simulink model "RBDmodel"  (R2023a)
settings: Solver=ode15s  StartTime=0.0  StopTime=4  FixedStep=0.0001  RelTol=1e-3  AbsTol=1e-3  EnableMultiTasking=on
model workspace (MAT data in the model file):
  C_Gimbal = 0.5
  C_IAP = 0.01
  IAP_Pa = 0
  K_Gimbal = 0
  K_IAP = 200
  LeftAbdominalMuscleForce = 0
  LeftBackMuscleForce = 0
  LeftTransverse1MuscleForce = 0
  LeftTransverse2MuscleForce = 0
  Moment_AR = 0
  Moment_FE = 7.5
  Moment_LB = 0
  RightAbdominalMuscleForce = 0
  RightBackMuscleForce = 0
  RightTransverse1MuscleForce = 0
  RightTransverse2MuscleForce = 0
  a = 1
  b = 1
  muscle_color = [0 0 1]
  muscle_radius = 1
undefined symbols (not defined in the file): X, Y, Z
libraries: nesl_utility x346, sm_lib x329, simulink_extras x33, checkpacklib x3, simulink x1
(part 5 of 12)

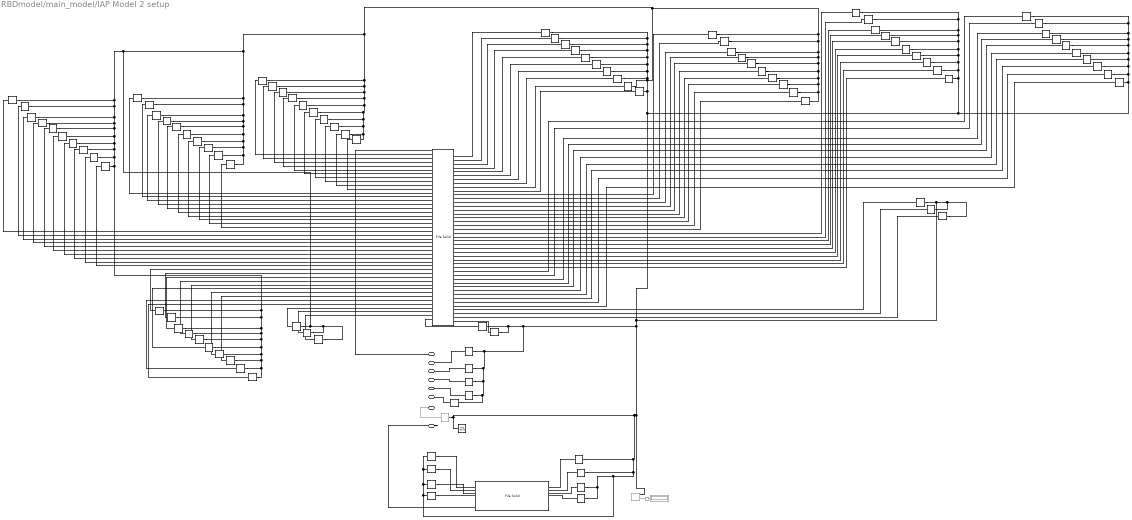
== system RBDmodel/main_model/IAP Model 2 setup ==
  Display : Display  Commented=on
  File Solid : sm_lib/Body Elements/File Solid  ExtGeomFileName=C:\Users\siril\OneDrive\Desktop\TIM-Control\Matlab\Simscape models\CAD - with COM\SymmetricModel\Abdominal COM Cone.step  UnitType=FromFile  ExtGeomFileUnits=m  StepReaderType=HEX  ExportConvexHullGeometry=off  InertiaType=CalculateFromGeometry  Mass=1  MassUnits=g  CenterOfMass=[0 0 0]  CenterOfMassUnits=m  MomentsOfInertia=[1 1 1]  MomentsOfInertiaUnits=kg*m^2  ProductsOfInertia=[0 0 0]  ProductsOfInertiaUnits=kg*m^2  BasedOnType=Density  Density=1000  DensityUnits=kg/m^3  DoExposeReferenceFrame=off  SerializedFrames=<Frames><Frame><Id>Frame1</Id><Value><Name>Abdominal COM</Name><Origin><Source>GeometricFeature</Source><FeatureName>point 8</FeatureName></Origin><PrimaryAxis><DefinedDirection>+Z</DefinedDirection><Source>ReferenceFrame</Source><SourceDirection>+Z</SourceDirection><FeatureName></FeatureName></PrimaryAxis><SecondaryAxis><DefinedDirection>+X</DefinedDirection><Source>ReferenceFrame</Source><SourceDirection>+X</SourceDirection><FeatureName></FeatureName></SecondaryAxis></Value></Frame></Frames>  GraphicType=FromGeometry  MarkerShape=Sphere  MarkerSize=10  GraphicVisPropType=SimpleVisualProperties  GraphicDiffuseColor=[1.0 0.2 0.2]  GraphicSpecularColor=[0.5 0.5 0.5 1.0]  GraphicAmbientColor=[0.15 0.15 0.15 1.0]  GraphicEmissiveColor=[0.0 0.0 0.0 1.0]  GraphicShininess=75  GraphicOpacity=1.0
  File Solid2 : sm_lib/Body Elements/File Solid  ExtGeomFileName=C:\Users\siril\OneDrive\Desktop\TIM-Control\Matlab\Simscape models\CAD - with COM\SymmetricModel\draft7\Abd-diamond-flat-solid.step  UnitType=FromFile  ExtGeomFileUnits=m  StepReaderType=HEX  ExportConvexHullGeometry=off  InertiaType=CalculateFromGeometry  Mass=1  MassUnits=kg  CenterOfMass=[0 0 0]  CenterOfMassUnits=m  MomentsOfInertia=[1 1 1]  MomentsOfInertiaUnits=kg*m^2  ProductsOfInertia=[0 0 0]  ProductsOfInertiaUnits=kg*m^2  BasedOnType=Density  Density=0.182  DensityUnits=g/cm^3  DoExposeReferenceFrame=on  SerializedFrames=<Frames><Frame><Id>Frame1</Id><Value><Name>To L1</Name><Origin><Source>GeometricFeature</Source><FeatureName>planar surface 723</FeatureName></Origin><PrimaryAxis><DefinedDirection>-Z</DefinedDirection><Source>GeometricFeature</Source><SourceDirection>+Z</SourceDirection><FeatureName>planar surface 723</FeatureName></PrimaryAxis><SecondaryAxis><DefinedDirection>+X</DefinedDirection><Source>ReferenceFrame</Source><SourceDirection>+X</SourceDirection><FeatureName></FeatureName></SecondaryAxis></Value></Frame><Frame><Id>Frame2</Id><Value><Name>L1</Name><Origin><Source>GeometricFeature</Source><FeatureName>planar surface 1442</FeatureName></Origin><PrimaryAxis><DefinedDirection>+Z</DefinedDirection><Source>GeometricFeature</Source><SourceDirection>+Z</SourceDirection><FeatureName>planar surface 1442</FeatureName></PrimaryAxis><SecondaryAxis><DefinedDirection>+X</DefinedDirection><Source>ReferenceFrame</Source><SourceDirection>+X</SourceDirection><FeatureName></FeatureName></SecondaryAxis></Value></Frame><Frame><Id>Frame3</Id><Value><Name>R1</Name><Origin><Source>GeometricFeature</Source><FeatureName>planar surface 707</FeatureName></Origin><PrimaryAxis><DefinedDirection>-Z</DefinedDirection><Source>GeometricFeature</Source><SourceDirection>+Z</SourceDirection><FeatureName>planar surface 707</FeatureName></PrimaryAxis><SecondaryAxis><DefinedDirection>+X</DefinedDirection><Source>ReferenceFrame</Source><SourceDirection>+X</SourceDirection><FeatureName></FeatureName></SecondaryAxis></Value></Frame><Frame><Id>Frame4</Id><Value><Name>L2</Name><Origin><Source>GeometricFeature</Source><FeatureName>planar surface 1450</FeatureName></Origin><PrimaryAxis><DefinedDirection>+Z</DefinedDirection><Source>GeometricFeature</Source><SourceDirection>+Z</SourceDirection><FeatureName>planar surface 1450</FeatureName></PrimaryAxis><SecondaryAxis><DefinedDirection>+X</DefinedDirection><Source>ReferenceFrame</Source><SourceDirection>+X</SourceDirection><FeatureName></FeatureName></SecondaryAxis></Value></Frame><Frame><Id>Frame5</Id><Value><Name>R2</Name><Origin><Source>GeometricFeature</Source><FeatureName>planar surface 715</FeatureName></Origin><PrimaryAxis><DefinedDirection>-Z</DefinedDirection><Source>GeometricFeature</Source><SourceDirection>+Z</SourceDirection><FeatureName>planar surface 715</FeatureName></PrimaryAxis><SecondaryAxis><DefinedDirection>+X</DefinedDirection><Source>ReferenceFrame</Source><SourceDirection>+X</SourceDirection><FeatureName></FeatureName></SecondaryAxis></Value></Frame><Frame><Id>Frame6</Id><Value><Name>L3</Name><Origin><Source>GeometricFeature</Source><FeatureName>planar surface 1412</FeatureName></Origin><PrimaryAxis><DefinedDirection>+Z</DefinedDirection><Source>GeometricFeature</Source><SourceDirection>+Z</SourceDirection><FeatureName>planar surface 1412</FeatureName></PrimaryAxis><SecondaryAxis><DefinedDirection>+X</DefinedDirection><Source>ReferenceFrame</Source><SourceDirection>+X</SourceDirection><FeatureName></FeatureName></SecondaryAxis></Value></Frame><Frame><Id>Frame7</Id><Value><Name>R3</Name><Origin><Source>GeometricFeature</Source><FeatureName>planar surface 677</FeatureName></Origin><PrimaryAxis><DefinedDirection>-Z</DefinedDirection><Source>GeometricFeature</Source><SourceDirection>+Z</SourceDirection><FeatureName>planar surface 677</FeatureName></PrimaryAxis><SecondaryAxis><DefinedDirection>+X</DefinedDirection><Source>ReferenceFrame</Source><SourceDirection>+X</SourceDirection><FeatureName></FeatureName></SecondaryAxis></Value></Frame><Frame><Id>Frame8</Id><Value><Name>L4</Name><Origin><Source>GeometricFeature</Source><FeatureName>planar surface 1159</FeatureName></Origin><PrimaryAxis><DefinedDirection>+Z</DefinedDirection><Source>GeometricFeature</Source><SourceDirection>+Z</SourceDirection><FeatureName>planar surface 1159</FeatureName></PrimaryAxis><SecondaryAxis><DefinedDirection>+X</DefinedDirection><Source>ReferenceFrame</Source><SourceDirection>+X</SourceDirection><FeatureName></FeatureName></SecondaryAxis></Value></Frame><Frame><Id>Frame9</Id><Value><Name>R4</Name><Origin><Source>GeometricFeature</Source><FeatureName>planar surface 431</FeatureName></Origin><PrimaryAxis><DefinedDirection>-Z</DefinedDirection><Source>GeometricFeature</Source><SourceDirection>+Z</SourceDirection><FeatureName>planar surface 431</FeatureName></PrimaryAxis><SecondaryAxis><DefinedDirection>+X</DefinedDirection><Source>ReferenceFrame</Source><SourceDirection>+X</SourceDirection><FeatureName></FeatureName></SecondaryAxis></Value></Frame><Frame><Id>Frame10</Id><Value><Name>L5</Name><Origin><Source>GeometricFeature</Source><FeatureName>planar surface 1433</FeatureName></Origin><PrimaryAxis><DefinedDirection>+Z</DefinedDirection><Source>GeometricFeature</Source><SourceDirection>+Z</SourceDirection><FeatureName>planar surface 1433</FeatureName></PrimaryAxis><SecondaryAxis><DefinedDirection>+X</DefinedDirection><Source>ReferenceFrame</Source><SourceDirection>+X</SourceDirection><FeatureName></FeatureName></SecondaryAxis></Value></Frame><Frame><Id>Frame11</Id><Value><Name>R5</Name><Origin><Source>GeometricFeature</Source><FeatureName>planar surface 698</FeatureName></Origin><PrimaryAxis><DefinedDirection>-Z</DefinedDirection><Source>GeometricFeature</Source><SourceDirection>+Z</SourceDirection><FeatureName>planar surface 698</FeatureName></PrimaryAxis><SecondaryAxis><DefinedDirection>+X</DefinedDirection><Source>ReferenceFrame</Source><SourceDirection>+X</SourceDirection><FeatureName></FeatureName></SecondaryAxis></Value></Frame><Frame><Id>Frame12</Id><Value><Name>L6</Name><Origin><Source>GeometricFeature</Source><FeatureName>planar surface 1135</FeatureName></Origin><PrimaryAxis><DefinedDirection>+Z</DefinedDirection><Source>GeometricFeature</Source><SourceDirection>+Z</SourceDirection><FeatureName>planar surface 1135</FeatureName></PrimaryAxis><SecondaryAxis><DefinedDirection>+X</DefinedDirection><Source>ReferenceFrame</Source><SourceDirection>+X</SourceDirection><FeatureName></FeatureName></SecondaryAxis></Value></Frame><Frame><Id>Frame13</Id><Value><Name>R6</Name><Origin><Source>GeometricFeature</Source><FeatureName>planar surface 407</FeatureName></Origin><PrimaryAxis><DefinedDirection>-Z</DefinedDirection><Source>GeometricFeature</Source><SourceDirection>+Z</SourceDirection><FeatureName>planar surface 407</FeatureName></PrimaryAxis><SecondaryAxis><DefinedDirection>+X</DefinedDirection><Source>ReferenceFrame</Source><SourceDirection>+X</SourceDirection><FeatureName></FeatureName></SecondaryAxis></Value></Frame><Frame><Id>Frame14</Id><Value><Name>L7</Name><Origin><Source>GeometricFeature</Source><FeatureName>planar surface 1217</FeatureName></Origin><PrimaryAxis><DefinedDirection>+Z</DefinedDirection><Source>GeometricFeature</Source><SourceDirection>+Z</SourceDirection><FeatureName>planar surface 1217</FeatureName></PrimaryAxis><SecondaryAxis><DefinedDirection>+X</DefinedDirection><Source>ReferenceFrame</Source><SourceDirection>+X</SourceDirection><FeatureName></FeatureName></SecondaryAxis></Value></Frame><Frame><Id>Frame15</Id><Value><Name>R7</Name><Origin><Source>GeometricFeature</Source><FeatureName>planar surface 482</FeatureName></Origin><PrimaryAxis><DefinedDirection>-Z</DefinedDirection><Source>GeometricFeature</Source><SourceDirection>+Z</SourceDirection><FeatureName>planar surface 482</FeatureName></PrimaryAxis><SecondaryAxis><DefinedDirection>+X</DefinedDirection><Source>ReferenceFrame</Source><SourceDirection>+X</SourceDirection><FeatureName></FeatureName></SecondaryAxis></Value></Frame><Frame><Id>Frame16</Id><Value><Name>L8</Name><Origin><Source>GeometricFeature</Source><FeatureName>planar surface 1125</FeatureName></Origin><PrimaryAxis><DefinedDirection>+Z</DefinedDirection><Source>GeometricFeature</Source><SourceDirection>+Z</SourceDirection><FeatureName>planar surface 1125</FeatureName></PrimaryAxis><SecondaryAxis><DefinedDirection>+X</DefinedDirection><Source>ReferenceFrame</Source><SourceDirection>+X</SourceDirection><FeatureName></FeatureName></SecondaryAxis></Value></Frame><Frame><Id>Frame17</Id><Value><Name>R8</Name><Origin><Source>GeometricFeature</Source><FeatureName>planar surface 397</FeatureName></Origin><PrimaryAxis><DefinedDirection>-Z</DefinedDirection><Source>GeometricFeature</Source><SourceDirection>+Z</SourceDirection><FeatureName>planar surface 397</FeatureName></PrimaryAxis><SecondaryAxis><DefinedDirection>+X</DefinedDirection><Source>ReferenceFrame</Source><SourceDirection>+X</SourceDirection><FeatureName></FeatureName></SecondaryAxis></Value></Frame><Frame><Id>Frame18</Id><Value><Name>L9</Name><Origin><Source>GeometricFeature</Source><FeatureName>planar surface 1123</FeatureName></Origin><PrimaryAxis><DefinedDirection>+Z</DefinedDirection><Source>GeometricFeature</Source><SourceDirection>+Z</SourceDirection><FeatureName>planar surface 1123</FeatureName></PrimaryAxis><SecondaryAxis><DefinedDirection>+X</DefinedDirection><Source>ReferenceFrame</Source><SourceDirection>+X</SourceDirection><FeatureName></FeatureName></SecondaryAxis></Value></Frame><Frame><Id>Frame19</Id><Value><Name>R9</Name><Origin><Source>GeometricFeature</Source><FeatureName>planar surface 395</FeatureName></Origin><PrimaryAxis><DefinedDirection>-Z</DefinedDirection><Source>GeometricFeature</Source><SourceDirection>+Z</SourceDirection><FeatureName>planar surface 395</FeatureName></PrimaryAxis><SecondaryAxis><DefinedDirection>+X</DefinedDirection><Source>ReferenceFrame</Source><SourceDirection>+X</SourceDirection><FeatureName></FeatureName></SecondaryAxis></Value></Frame><Frame><Id>Frame20</Id><Value><Name>L10</Name><Origin><Source>GeometricFeature</Source><FeatureName>planar surface 1120</FeatureName></Origin><PrimaryAxis><DefinedDirection>+Z</DefinedDirection><Source>GeometricFeature</Source><SourceDirection>+Z</SourceDirection><FeatureName>planar surface 1120</FeatureName></PrimaryAxis><SecondaryAxis><DefinedDirection>+X</DefinedDirection><Source>ReferenceFrame</Source><SourceDirection>+X</SourceDirection><FeatureName></FeatureName></SecondaryAxis></Value></Frame><Frame><Id>Frame21</Id><Value><Name>R10</Name><Origin><Source>GeometricFeature</Source><FeatureName>planar surface 392</FeatureName></Origin><PrimaryAxis><DefinedDirection>-Z</DefinedDirection><Source>GeometricFeature</Source><SourceDirection>+Z</SourceDirection><FeatureName>planar surface 392</FeatureName></PrimaryAxis><SecondaryAxis><DefinedDirection>+X</DefinedDirection><Source>ReferenceFrame</Source><SourceDirection>+X</SourceDirection><FeatureName></FeatureName></SecondaryAxis></Value></Frame><Frame><Id>Frame22</Id><Value><Name>L11</Name><Origin><Source>GeometricFeature</Source><FeatureName>planar surface 1182</FeatureName></Origin><PrimaryAxis><DefinedDirection>+Z</DefinedDirection><Source>GeometricFeature</Source><SourceDirection>+Z</SourceDirection><FeatureName>planar surface 1182</FeatureName></PrimaryAxis><SecondaryAxis><DefinedDirection>+X</DefinedDirection><Source>ReferenceFrame</Source><SourceDirection>+X</SourceDirection><FeatureName></FeatureName></SecondaryAxis></Value></Frame><Frame><Id>Frame23</Id><Value><Name>R11</Name><Origin><Source>GeometricFeature</Source><FeatureName>planar surface 452</FeatureName></Origin><PrimaryAxis><DefinedDirection>-Z</DefinedDirection><Source>GeometricFeature</Source><SourceDirection>+Z</SourceDirection><FeatureName>planar surface 452</FeatureName></PrimaryAxis><SecondaryAxis><DefinedDirection>+X</DefinedDirection><Source>ReferenceFrame</Source><SourceDirection>+X</SourceDirection><FeatureName></FeatureName></SecondaryAxis></Value></Frame><Frame><Id>Frame24</Id><Value><Name>L12</Name><Origin><Source>GeometricFeature</Source><FeatureName>planar surface 1305</FeatureName></Origin><PrimaryAxis><DefinedDirection>+Z</DefinedDirection><Source>GeometricFeature</Source><SourceDirection>+Z</SourceDirection><FeatureName>planar surface 1305</FeatureName></PrimaryAxis><SecondaryAxis><DefinedDirection>+X</DefinedDirection><Source>ReferenceFrame</Source><SourceDirection>+X</SourceDirection><FeatureName></FeatureName></SecondaryAxis></Value></Frame><Frame><Id>Frame25</Id><Value><Name>R12</Name><Origin><Source>GeometricFeature</Source><FeatureName>planar surface 570</FeatureName></Origin><PrimaryAxis><DefinedDirection>-Z</DefinedDirection><Source>GeometricFeature</Source><SourceDirection>+Z</SourceDirection><FeatureName>planar surface 570</FeatureName></PrimaryAxis><SecondaryAxis><DefinedDirection>+X</DefinedDirection><Source>ReferenceFrame</Source><SourceDirection>+X</SourceDirection><FeatureName></FeatureName></SecondaryAxis></Value></Frame><Frame><Id>Frame26</Id><Value><Name>L13</Name><Origin><Source>GeometricFeature</Source><FeatureName>planar surface 1216</FeatureName></Origin><PrimaryAxis><DefinedDirection>+Z</DefinedDirection><Source>GeometricFeature</Source><SourceDirection>+Z</SourceDirection><FeatureName>planar surface 1216</FeatureName></PrimaryAxis><SecondaryAxis><DefinedDirection>+X</DefinedDirection><Source>ReferenceFrame</Source><SourceDirection>+X</SourceDirection><FeatureName></FeatureName></SecondaryAxis></Value></Frame><Frame><Id>Frame27</Id><Value><Name>R13</Name><Origin><Source>GeometricFeature</Source><FeatureName>planar surface 481</FeatureName></Origin><PrimaryAxis><DefinedDirection>-Z</DefinedDirection><Source>GeometricFeature</Source><SourceDirection>+Z</SourceDirection><FeatureName>planar surface 481</FeatureName></PrimaryAxis><SecondaryAxis><DefinedDirection>+X</DefinedDirection><Source>ReferenceFrame</Source><SourceDirection>+X</SourceDirection><FeatureName></FeatureName></SecondaryAxis></Value></Frame><Frame><Id>Frame28</Id><Value><Name>L14</Name><Origin><Source>GeometricFeature</Source><FeatureName>planar surface 1062</FeatureName></Origin><PrimaryAxis><DefinedDirection>+Z</DefinedDirection><Source>GeometricFeature</Source><SourceDirection>+Z</SourceDirection><FeatureName>planar surface 1062</FeatureName></PrimaryAxis><SecondaryAxis><DefinedDirection>+X</DefinedDirection><Source>ReferenceFrame</Source><SourceDirection>+X</SourceDirection><FeatureName></FeatureName></SecondaryAxis></Value></Frame><Frame><Id>Frame29</Id><Value><Name>R14</Name><Origin><Source>GeometricFeature</Source><FeatureName>planar surface 334</FeatureName></Origin><PrimaryAxis><DefinedDirection>-Z</DefinedDirection><Source>GeometricFeature</Source><SourceDirection>+Z</SourceDirection><FeatureName>planar surface 334</FeatureName></PrimaryAxis><SecondaryAxis><DefinedDirection>+X</DefinedDirection><Source>ReferenceFrame</Source><SourceDirection>+X</SourceDirection><FeatureName></FeatureName></SecondaryAxis></Value></Frame><Frame><Id>Frame30</Id><Value><Name>L15</Name><Origin><Source>GeometricFeature</Source><FeatureName>planar surface 1242</FeatureName></Origin><PrimaryAxis><DefinedDirection>+Z</DefinedDirection><Source>GeometricFeature</Source><SourceDirection>+Z</SourceDirection><FeatureName>planar surface 1242</FeatureName></PrimaryAxis><SecondaryAxis><DefinedDirection>+X</DefinedDirection><Source>ReferenceFrame</Source><SourceDirection>+X</SourceDirection><FeatureName></FeatureName></SecondaryAxis></Value></Frame><Frame><Id>Frame31</Id><Value><Name>R15</Name><Origin><Source>GeometricFeature</Source><FeatureName>planar surface 507</FeatureName></Origin><PrimaryAxis><DefinedDirection>-Z</DefinedDirection><Source>GeometricFeature</Source><SourceDirection>+Z</SourceDirection><FeatureName>planar surface 507</FeatureName></PrimaryAxis><SecondaryAxis><DefinedDirection>+X</DefinedDirection><Source>ReferenceFrame</Source><SourceDirection>+X</SourceDirection><FeatureName></FeatureName></SecondaryAxis></Value></Frame><Frame><Id>Frame32</Id><Value><Name>L16</Name><Origin><Source>GeometricFeature</Source><FeatureName>planar surface 1026</FeatureName></Origin><PrimaryAxis><DefinedDirection>+Z</DefinedDirection><Source>GeometricFeature</Source><SourceDirection>+Z</SourceDirection><FeatureName>planar surface 1026</FeatureName></PrimaryAxis><SecondaryAxis><DefinedDirection>+X</DefinedDirection><Source>ReferenceFrame</Source><SourceDirection>+X</SourceDirection><FeatureName></FeatureName></SecondaryAxis></Value></Frame><Frame><Id>Frame33</Id><Value><Name>R16</Name><Origin><Source>GeometricFeature</Source><FeatureName>planar surface 298</FeatureName></Origin><PrimaryAxis><DefinedDirection>-Z</DefinedDirection><Source>GeometricFeature</Source><SourceDirection>+Z</SourceDirection><FeatureName>planar surface 298</FeatureName></PrimaryAxis><SecondaryAxis><DefinedDirection>+X</DefinedDirection><Source>ReferenceFrame</Source><SourceDirection>+X</SourceDirection><FeatureName></FeatureName></SecondaryAxis></Value></Frame><Frame><Id>Frame34</Id><Value><Name>L17</Name><Origin><Source>GeometricFeature</Source><FeatureName>planar surface 1339</FeatureName></Origin><PrimaryAxis><DefinedDirection>+Z</DefinedDirection><Source>GeometricFeature</Source><SourceDirection>+Z</SourceDirection><FeatureName>planar surface 1339</FeatureName></PrimaryAxis><SecondaryAxis><DefinedDirection>+X</DefinedDirection><Source>ReferenceFrame</Source><SourceDirection>+X</SourceDirection><FeatureName></FeatureName></SecondaryAxis></Value></Frame><Frame><Id>Frame35</Id><Value><Name>R17</Name><Origin><Source>GeometricFeature</Source><FeatureName>planar surface 604</FeatureName></Origin><PrimaryAxis><DefinedDirection>-Z</DefinedDirection><Source>GeometricFeature</Source><SourceDirection>+Z</SourceDirection><FeatureName>planar surface 604</FeatureName></PrimaryAxis><SecondaryAxis><DefinedDirection>+X</DefinedDirection><Source>ReferenceFrame</Source><SourceDirection>+X</SourceDirection><FeatureName></FeatureName></SecondaryAxis></Value></Frame><Frame><Id>Frame36</Id><Value><Name>L18</Name><Origin><Source>GeometricFeature</Source><FeatureName>planar surface 1004</FeatureName></Origin><PrimaryAxis><DefinedDirection>+Z</DefinedDirection><Source>GeometricFeature</Source><SourceDirection>+Z</SourceDirection><FeatureName>planar surface 1004</FeatureName></PrimaryAxis><SecondaryAxis><DefinedDirection>+X</DefinedDirection><Source>ReferenceFrame</Source><SourceDirection>+X</SourceDirection><FeatureName></FeatureName></SecondaryAxis></Value></Frame><Frame><Id>Frame37</Id><Value><Name>R18</Name><Origin><Source>GeometricFeature</Source><FeatureName>planar surface 276</FeatureName></Origin><PrimaryAxis><DefinedDirection>-Z</DefinedDirection><Source>GeometricFeature</Source><SourceDirection>+Z</SourceDirection><FeatureName>planar surface 276</FeatureName></PrimaryAxis><SecondaryAxis><DefinedDirection>+X</DefinedDirection><Source>ReferenceFrame</Source><SourceDirection>+X</SourceDirection><FeatureName></FeatureName></SecondaryAxis></Value></Frame><Frame><Id>Frame38</Id><Value><Name>L19</Name><Origin><Source>GeometricFeature</Source><FeatureName>planar surface 996</FeatureName></Origin><PrimaryAxis><DefinedDirection>+Z</DefinedDirection><Source>GeometricFeature</Source><SourceDirection>+Z</SourceDirection><FeatureName>planar surface 996</FeatureName></PrimaryAxis><SecondaryAxis><DefinedDirection>+X</DefinedDirection><Source>ReferenceFrame</Source><SourceDirection>+X</SourceDirection><FeatureName></FeatureName></SecondaryAxis></Value></Frame><Frame><Id>Frame39</Id><Value><Name>R19</Name><Origin><Source>GeometricFeature</Source><FeatureName>planar surface 268</FeatureName></Origin><PrimaryAxis><DefinedDirection>-Z</DefinedDirection><Source>GeometricFeature</Source><SourceDirection>+Z</SourceDirection><FeatureName>planar surface 268</FeatureName></PrimaryAxis><SecondaryAxis><DefinedDirection>+X</DefinedDirection><Source>ReferenceFrame</Source><SourceDirection>+X</SourceDirection><FeatureName></FeatureName></SecondaryAxis></Value></Frame><Frame><Id>Frame40</Id><Value><Name>L20</Name><Origin><Source>GeometricFeature</Source><FeatureName>planar surface 987</FeatureName></Origin><PrimaryAxis><DefinedDirection>+Z</DefinedDirection><Source>GeometricFeature</Source><SourceDirection>+Z</SourceDirection><FeatureName>planar surface 987</FeatureName></PrimaryAxis><SecondaryAxis><DefinedDirection>+X</DefinedDirection><Source>ReferenceFrame</Source><SourceDirection>+X</SourceDirection><FeatureName></FeatureName></SecondaryAxis></Value></Frame><Frame><Id>Frame41</Id><Value><Name>R20</Name><Origin><Source>GeometricFeature</Source><FeatureName>planar surface 259</FeatureName></Origin><PrimaryAxis><DefinedDirection>-Z</DefinedDirection><Source>GeometricFeature</Source><SourceDirection>+Z</SourceDirection><FeatureName>planar surface 259</FeatureName></PrimaryAxis><SecondaryAxis><DefinedDirection>+X</DefinedDirection><Source>ReferenceFrame</Source><SourceDirection>+X</SourceDirection><FeatureName></FeatureName></SecondaryAxis></Value></Frame><Frame><Id>Frame42</Id><Value><Name>L21</Name><Origin><Source>GeometricFeature</Source><FeatureName>planar surface 1218</FeatureName></Origin><PrimaryAxis><DefinedDirection>+Z</DefinedDirection><Source>GeometricFeature</Source><SourceDirection>+Z</SourceDirection><FeatureName>planar surface 1218</FeatureName></PrimaryAxis><SecondaryAxis><DefinedDirection>+X</DefinedDirection><Source>ReferenceFrame</Source><SourceDirection>+X</SourceDirection><FeatureName></FeatureName></SecondaryAxis></Value></Frame><Frame><Id>Frame43</Id><Value><Name>R21</Name><Origin><Source>GeometricFeature</Source><FeatureName>planar surface 483</FeatureName></Origin><PrimaryAxis><DefinedDirection>-Z</DefinedDirection><Source>GeometricFeature</Source><SourceDirection>+Z</SourceDirection><FeatureName>planar surface 483</FeatureName></PrimaryAxis><SecondaryAxis><DefinedDirection>+X</DefinedDirection><Source>ReferenceFrame</Source><SourceDirection>+X</SourceDirection><FeatureName></FeatureName></SecondaryAxis></Value></Frame><Frame><Id>Frame44</Id><Value><Name>L22</Name><Origin><Source>GeometricFeature</Source><FeatureName>planar surface 1364</FeatureName></Origin><PrimaryAxis><DefinedDirection>+Z</DefinedDirection><Source>GeometricFeature</Source><SourceDirection>+Z</SourceDirection><FeatureName>planar surface 1364</FeatureName></PrimaryAxis><SecondaryAxis><DefinedDirection>+X</DefinedDirection><Source>ReferenceFrame</Source><SourceDirection>+X</SourceDirection><FeatureName></FeatureName></SecondaryAxis></Value></Frame><Frame><Id>Frame45</Id><Value><Name>R22</Name><Origin><Source>GeometricFeature</Source><FeatureName>planar surface 629</FeatureName></Origin><PrimaryAxis><DefinedDirection>-Z</DefinedDirection><Source>GeometricFeature</Source><SourceDirection>+Z</SourceDirection><FeatureName>planar surface 629</FeatureName></PrimaryAxis><SecondaryAxis><DefinedDirection>+X</DefinedDirection><Source>ReferenceFrame</Source><SourceDirection>+X</SourceDirection><FeatureName></FeatureName></SecondaryAxis></Value></Frame><Frame><Id>Frame46</Id><Value><Name>L23</Name><Origin><Source>GeometricFeature</Source><FeatureName>planar surface 1381</FeatureName></Origin><PrimaryAxis><DefinedDirection>+Z</DefinedDirection><Source>GeometricFeature</Source><SourceDirection>+Z</SourceDirection><FeatureName>planar surface 1381</FeatureName></PrimaryAxis><SecondaryAxis><DefinedDirection>+X</DefinedDirection><Source>ReferenceFrame</Source><SourceDirection>+X</SourceDirection><FeatureName></FeatureName></SecondaryAxis></Value></Frame><Frame><Id>Frame47</Id><Value><Name>R23</Name><Origin><Source>GeometricFeature</Source><FeatureName>planar surface 646</FeatureName></Origin><PrimaryAxis><DefinedDirection>-Z</DefinedDirection><Source>GeometricFeature</Source><SourceDirection>+Z</SourceDirection><FeatureName>planar surface 646</FeatureName></PrimaryAxis><SecondaryAxis><DefinedDirection>+X</DefinedDirection><Source>ReferenceFrame</Source><SourceDirection>+X</SourceDirection><FeatureName></FeatureName></SecondaryAxis></Value></Frame><Frame><Id>Frame48</Id><Value><Name>L24</Name><Origin><Source>GeometricFeature</Source><FeatureName>planar surface 950</FeatureName></Origin><PrimaryAxis><DefinedDirection>+Z</DefinedDirection><Source>GeometricFeature</Source><SourceDirection>+Z</SourceDirection><FeatureName>planar surface 950</FeatureName></PrimaryAxis><SecondaryAxis><DefinedDirection>+X</DefinedDirection><Source>ReferenceFrame</Source><SourceDirection>+X</SourceDirection><FeatureName></FeatureName></SecondaryAxis></Value></Frame><Frame><Id>Frame49</Id><Value><Name>R24</Name><Origin><Source>GeometricFeature</Source><FeatureName>planar surface 222</FeatureName></Origin><PrimaryAxis><DefinedDirection>-Z</DefinedDirection><Source>GeometricFeature</Source><SourceDirection>+Z</SourceDirection><FeatureName>planar surface 222</FeatureName></PrimaryAxis><SecondaryAxis><DefinedDirection>+X</DefinedDirection><Source>ReferenceFrame</Source><SourceDirection>+X</SourceDirection><FeatureName></FeatureName></SecondaryAxis></Value></Frame><Frame><Id>Frame50</Id><Value><Name>L25</Name><Origin><Source>GeometricFeature</Source><FeatureName>planar surface 1231</FeatureName></Origin><PrimaryAxis><DefinedDirection>+Z</DefinedDirection><Source>GeometricFeature</Source><SourceDirection>+Z</SourceDirection><FeatureName>planar surface 1231</FeatureName></PrimaryAxis><SecondaryAxis><DefinedDirection>+X</DefinedDirection><Source>ReferenceFrame</Source><SourceDirection>+X</SourceDirection><FeatureName></FeatureName></SecondaryAxis></Value></Frame><Frame><Id>Frame51</Id><Value><Name>R25</Name><Origin><Source>GeometricFeature</Source><FeatureName>planar surface 496</FeatureName></Origin><PrimaryAxis><DefinedDirection>-Z</DefinedDirection><Source>GeometricFeature</Source><SourceDirection>+Z</SourceDirection><FeatureName>planar surface 496</FeatureName></PrimaryAxis><SecondaryAxis><DefinedDirection>+X</DefinedDirection><Source>ReferenceFrame</Source><SourceDirection>+X</SourceDirection><FeatureName></FeatureName></SecondaryAxis></Value></Frame><Frame><Id>Frame52</Id><Value><Name>L26</Name><Origin><Source>GeometricFeature</Source><FeatureName>planar surface 916</FeatureName></Origin><PrimaryAxis><DefinedDirection>+Z</DefinedDirection><Source>GeometricFeature</Source><SourceDirection>+Z</SourceDirection><FeatureName>planar surface 916</FeatureName></PrimaryAxis><SecondaryAxis><DefinedDirection>+X</DefinedDirection><Source>ReferenceFrame</Source><SourceDirection>+X</SourceDirection><FeatureName></FeatureName></SecondaryAxis></Value></Frame><Frame><Id>Frame53</Id><Value><Name>R26</Name><Origin><Source>GeometricFeature</Source><FeatureName>planar surface 188</FeatureName></Origin><PrimaryAxis><DefinedDirection>-Z</DefinedDirection><Source>GeometricFeature</Source><SourceDirection>+Z</SourceDirection><FeatureName>planar surface 188</FeatureName></PrimaryAxis><SecondaryAxis><DefinedDirection>+X</DefinedDirection><Source>ReferenceFrame</Source><SourceDirection>+X</SourceDirection><FeatureName></FeatureName></SecondaryAxis></Value></Frame><Frame><Id>Frame54</Id><Value><Name>L27</Name><Origin><Source>GeometricFeature</Source><FeatureName>planar surface 1358</FeatureName></Origin><PrimaryAxis><DefinedDirection>+Z</DefinedDirection><Source>GeometricFeature</Source><SourceDirection>+Z</SourceDirection><FeatureName>planar surface 1358</FeatureName></PrimaryAxis><SecondaryAxis><DefinedDirection>+X</DefinedDirection><Source>ReferenceFrame</Source><SourceDirection>+X</SourceDirection><FeatureName></FeatureName></SecondaryAxis></Value></Frame><Frame><Id>Frame55</Id><Value><Name>R27</Name><Origin><Source>GeometricFeature</Source><FeatureName>planar surface 623</FeatureName></Origin><PrimaryAxis><DefinedDirection>-Z</DefinedDirection><Source>GeometricFeature</Source><SourceDirection>+Z</SourceDirection><FeatureName>planar surface 623</FeatureName></PrimaryAxis><SecondaryAxis><DefinedDirection>+X</DefinedDirection><Source>ReferenceFrame</Source><SourceDirection>+X</SourceDirection><FeatureName></FeatureName></SecondaryAxis></Value></Frame><Frame><Id>Frame56</Id><Value><Name>L28</Name><Origin><Source>GeometricFeature</Source><FeatureName>planar surface 896</FeatureName></Origin><PrimaryAxis><DefinedDirection>+Z</DefinedDirection><Source>GeometricFeature</Source><SourceDirection>+Z</SourceDirection><FeatureName>planar surface 896</FeatureName></PrimaryAxis><SecondaryAxis><DefinedDirection>+X</DefinedDirection><Source>ReferenceFrame</Source><SourceDirection>+X</SourceDirection><FeatureName></FeatureName></SecondaryAxis></Value></Frame><Frame><Id>Frame57</Id><Value><Name>R28</Name><Origin><Source>GeometricFeature</Source><FeatureName>planar surface 168</FeatureName></Origin><PrimaryAxis><DefinedDirection>-Z</DefinedDirection><Source>GeometricFeature</Source><SourceDirection>+Z</SourceDirection><FeatureName>planar surface 168</FeatureName></PrimaryAxis><SecondaryAxis><DefinedDirection>+X</DefinedDirection><Source>ReferenceFrame</Source><SourceDirection>+X</SourceDirection><FeatureName></FeatureName></SecondaryAxis></Value></Frame><Frame><Id>Frame58</Id><Value><Name>L29</Name><Origin><Source>GeometricFeature</Source><FeatureName>planar surface 889</FeatureName></Origin><PrimaryAxis><DefinedDirection>+Z</DefinedDirection><Source>GeometricFeature</Source><SourceDirection>+Z</SourceDirection><FeatureName>planar surface 889</FeatureName></PrimaryAxis><SecondaryAxis><DefinedDirection>+X</DefinedDirection><Source>ReferenceFrame</Source><SourceDirection>+X</SourceDirection><FeatureName></FeatureName></SecondaryAxis></Value></Frame><Frame><Id>Frame59</Id><Value><Name>R29</Name><Origin><Source>GeometricFeature</Source><FeatureName>planar surface 161</FeatureName></Origin><PrimaryAxis><DefinedDirection>-Z</DefinedDirection><Source>GeometricFeature</Source><SourceDirection>+Z</SourceDirection><FeatureName>planar surface 161</FeatureName></PrimaryAxis><SecondaryAxis><DefinedDirection>+X</DefinedDirection><Source>ReferenceFrame</Source><SourceDirection>+X</SourceDirection><FeatureName></FeatureName></SecondaryAxis></Value></Frame><Frame><Id>Frame60</Id><Value><Name>L30</Name><Origin><Source>GeometricFeature</Source><FeatureName>planar surface 881</FeatureName></Origin><PrimaryAxis><DefinedDirection>+Z</DefinedDirection><Source>GeometricFeature</Source><SourceDirection>+Z</SourceDirection><FeatureName>planar surface 881</FeatureName></PrimaryAxis><SecondaryAxis><DefinedDirection>+X</DefinedDirection><Source>ReferenceFrame</Source><SourceDirection>+X</SourceDirection><FeatureName></FeatureName></SecondaryAxis></Value></Frame><Frame><Id>Frame61</Id><Value><Name>R30</Name><Origin><Source>GeometricFeature</Source><FeatureName>planar surface 153</FeatureName></Origin><PrimaryAxis><DefinedDirection>-Z</DefinedDirection><Source>GeometricFeature</Source><SourceDirection>+Z</SourceDirection><FeatureName>planar surface 153</FeatureName></PrimaryAxis><SecondaryAxis><DefinedDirection>+X</DefinedDirection><Source>ReferenceFrame</Source><SourceDirection>+X</SourceDirection><FeatureName></FeatureName></SecondaryAxis></Value></Frame><Frame><Id>Frame62</Id><Value><Name>L31</Name><Origin><Source>GeometricFeature</Source><FeatureName>planar surface 1280</FeatureName></Origin><PrimaryAxis><DefinedDirection>+Z</DefinedDirection><Source>GeometricFeature</Source><SourceDirection>+Z</SourceDirection><FeatureName>planar surface 1280</FeatureName></PrimaryAxis><SecondaryAxis><DefinedDirection>+X</DefinedDirection><Source>ReferenceFrame</Source><SourceDirection>+X</SourceDirection><FeatureName></FeatureName></SecondaryAxis></Value></Frame><Frame><Id>Frame63</Id><Value><Name>R31</Name><Origin><Source>GeometricFeature</Source><FeatureName>planar surface 545</FeatureName></Origin><PrimaryAxis><DefinedDirection>-Z</DefinedDirection><Source>GeometricFeature</Source><SourceDirection>+Z</SourceDirection><FeatureName>planar surface 545</FeatureName></PrimaryAxis><SecondaryAxis><DefinedDirection>+X</DefinedDirection><Source>ReferenceFrame</Source><SourceDirection>+X</SourceDirection><FeatureName></FeatureName></SecondaryAxis></Value></Frame><Frame><Id>Frame64</Id><Value><Name>L32</Name><Origin><Source>GeometricFeature</Source><FeatureName>planar surface 1224</FeatureName></Origin><PrimaryAxis><DefinedDirection>+Z</DefinedDirection><Source>GeometricFeature</Source><SourceDirection>+Z</SourceDirection><FeatureName>planar surface 1224</FeatureName></PrimaryAxis><SecondaryAxis><DefinedDirection>+X</DefinedDirection><Source>ReferenceFrame</Source><SourceDirection>+X</SourceDirection><FeatureName></FeatureName></SecondaryAxis></Value></Frame><Frame><Id>Frame65</Id><Value><Name>R32</Name><Origin><Source>GeometricFeature</Source><FeatureName>planar surface 489</FeatureName></Origin><PrimaryAxis><DefinedDirection>-Z</DefinedDirection><Source>GeometricFeature</Source><SourceDirection>+Z</SourceDirection><FeatureName>planar surface 489</FeatureName></PrimaryAxis><SecondaryAxis><DefinedDirection>+X</DefinedDirection><Source>ReferenceFrame</Source><SourceDirection>+X</SourceDirection><FeatureName></FeatureName></SecondaryAxis></Value></Frame><Frame><Id>Frame66</Id><Value><Name>L33</Name><Origin><Source>GeometricFeature</Source><FeatureName>planar surface 1400</FeatureName></Origin><PrimaryAxis><DefinedDirection>+Z</DefinedDirection><Source>GeometricFeature</Source><SourceDirection>+Z</SourceDirection><FeatureName>planar surface 1400</FeatureName></PrimaryAxis><SecondaryAxis><DefinedDirection>+X</DefinedDirection><Source>ReferenceFrame</Source><SourceDirection>+X</SourceDirection><FeatureName></FeatureName></SecondaryAxis></Value></Frame><Frame><Id>Frame67</Id><Value><Name>R33</Name><Origin><Source>GeometricFeature</Source><FeatureName>planar surface 665</FeatureName></Origin><PrimaryAxis><DefinedDirection>-Z</DefinedDirection><Source>GeometricFeature</Source><SourceDirection>+Z</SourceDirection><FeatureName>planar surface 665</FeatureName></PrimaryAxis><SecondaryAxis><DefinedDirection>+X</DefinedDirection><Source>ReferenceFrame</Source><SourceDirection>+X</SourceDirection><FeatureName></FeatureName></SecondaryAxis></Value></Frame><Frame><Id>Frame68</Id><Value><Name>L34</Name><Origin><Source>GeometricFeature</Source><FeatureName>planar surface 848</FeatureName></Origin><PrimaryAxis><DefinedDirection>+Z</DefinedDirection><Source>GeometricFeature</Source><SourceDirection>+Z</SourceDirection><FeatureName>planar surface 848</FeatureName></PrimaryAxis><SecondaryAxis><DefinedDirection>+X</DefinedDirection><Source>ReferenceFrame</Source><SourceDirection>+X</SourceDirection><FeatureName></FeatureName></SecondaryAxis></Value></Frame><Frame><Id>Frame69</Id><Value><Name>R34</Name><Origin><Source>GeometricFeature</Source><FeatureName>planar surface 120</FeatureName></Origin><PrimaryAxis><DefinedDirection>-Z</DefinedDirection><Source>GeometricFeature</Source><SourceDirection>+Z</SourceDirection><FeatureName>planar surface 120</FeatureName></PrimaryAxis><SecondaryAxis><DefinedDirection>+X</DefinedDirection><Source>ReferenceFrame</Source><SourceDirection>+X</SourceDirection><FeatureName></FeatureName></SecondaryAxis></Value></Frame><Frame><Id>Frame70</Id><Value><Name>L35</Name><Origin><Source>GeometricFeature</Source><FeatureName>planar surface 1385</FeatureName></Origin><PrimaryAxis><DefinedDirection>+Z</DefinedDirection><Source>GeometricFeature</Source><SourceDirection>+Z</SourceDirection><FeatureName>planar surface 1385</FeatureName></PrimaryAxis><SecondaryAxis><DefinedDirection>+X</DefinedDirection><Source>ReferenceFrame</Source><SourceDirection>+X</SourceDirection><FeatureName></FeatureName></SecondaryAxis></Value></Frame><Frame><Id>Frame71</Id><Value><Name>R35</Name><Origin><Source>GeometricFeature</Source><FeatureName>planar surface 650</FeatureName></Origin><PrimaryAxis><DefinedDirection>-Z</DefinedDirection><Source>GeometricFeature</Source><SourceDirection>+Z</SourceDirection><FeatureName>planar surface 650</FeatureName></PrimaryAxis><SecondaryAxis><DefinedDirection>+X</DefinedDirection><Source>ReferenceFrame</Source><SourceDirection>+X</SourceDirection><FeatureName></FeatureName></SecondaryAxis></Value></Frame><Frame><Id>Frame72</Id><Value><Name>L36</Name><Origin><Source>GeometricFeature</Source><FeatureName>planar surface 816</FeatureName></Origin><PrimaryAxis><DefinedDirection>+Z</DefinedDirection><Source>GeometricFeature</Source><SourceDirection>+Z</SourceDirection><FeatureName>planar surface 816</FeatureName></PrimaryAxis><SecondaryAxis><DefinedDirection>+X</DefinedDirection><Source>ReferenceFrame</Source><SourceDirection>+X</SourceDirection><FeatureName></FeatureName></SecondaryAxis></Value></Frame><Frame><Id>Frame73</Id><Value><Name>R36</Name><Origin><Source>GeometricFeature</Source><FeatureName>planar surface 88</FeatureName></Origin><PrimaryAxis><DefinedDirection>-Z</DefinedDirection><Source>GeometricFeature</Source><SourceDirection>+Z</SourceDirection><FeatureName>planar surface 88</FeatureName></PrimaryAxis><SecondaryAxis><DefinedDirection>+X</DefinedDirection><Source>ReferenceFrame</Source><SourceDirection>+X</SourceDirection><FeatureName></FeatureName></SecondaryAxis></Value></Frame><Frame><Id>Frame74</Id><Value><Name>L37</Name><Origin><Source>GeometricFeature</Source><FeatureName>segment 6127</FeatureName></Origin><PrimaryAxis><DefinedDirection>+Z</DefinedDirection><Source>GeometricFeature</Source><SourceDirection>+Z</SourceDirection><FeatureName>segment 6128</FeatureName></PrimaryAxis><SecondaryAxis><DefinedDirection>+X</DefinedDirection><Source>ReferenceFrame</Source><SourceDirection>+X</SourceDirection><FeatureName></FeatureName></SecondaryAxis></Value></Frame><Frame><Id>Frame75</Id><Value><Name>R37</Name><Origin><Source>GeometricFeature</Source><FeatureName>segment 6112</FeatureName></Origin><PrimaryAxis><DefinedDirection>+Z</DefinedDirection><Source>GeometricFeature</Source><SourceDirection>+Z</SourceDirection><FeatureName>segment 6123</FeatureName></PrimaryAxis><SecondaryAxis><DefinedDirection>+X</DefinedDirection><Source>ReferenceFrame</Source><SourceDirection>+X</SourceDirection><FeatureName></FeatureName></SecondaryAxis></Value></Frame><Frame><Id>Frame76</Id><Value><Name>L38</Name><Origin><Source>GeometricFeature</Source><FeatureName>segment 6294</FeatureName></Origin><PrimaryAxis><DefinedDirection>+Z</DefinedDirection><Source>GeometricFeature</Source><SourceDirection>+Z</SourceDirection><FeatureName>segment 6289</FeatureName></PrimaryAxis><SecondaryAxis><DefinedDirection>+Y</DefinedDirection><Source>ReferenceFrame</Source><SourceDirection>+X</SourceDirection><FeatureName></FeatureName></SecondaryAxis></Value></Frame><Frame><Id>Frame77</Id><Value><Name>R38</Name><Origin><Source>GeometricFeature</Source><FeatureName>segment 6267</FeatureName></Origin><PrimaryAxis><DefinedDirection>+Z</DefinedDirection><Source>GeometricFeature</Source><SourceDirection>+Z</SourceDirection><FeatureName>segment 6282</FeatureName></PrimaryAxis><SecondaryAxis><DefinedDirection>-Y</DefinedDirection><Source>ReferenceFrame</Source><SourceDirection>+X</SourceDirection><FeatureName></FeatureName></SecondaryAxis></Value></Frame><Frame><Id>Frame78</Id><Value><Name>L39</Name><Origin><Source>GeometricFeature</Source><FeatureName>segment 6303</FeatureName></Origin><PrimaryAxis><DefinedDirection>+Z</DefinedDirection><Source>GeometricFeature</Source><SourceDirection>+Z</SourceDirection><FeatureName>segment 6469</FeatureName></PrimaryAxis><SecondaryAxis><DefinedDirection>-Y</DefinedDirection><Source>ReferenceFrame</Source><SourceDirection>+X</SourceDirection><FeatureName></FeatureName></SecondaryAxis></Value></Frame><Frame><Id>Frame79</Id><Value><Name>R39</Name><Origin><Source>GeometricFeature</Source><FeatureName>segment 6263</FeatureName></Origin><PrimaryAxis><DefinedDirection>+Z</DefinedDirection><Source>GeometricFeature</Source><SourceDirection>+Z</SourceDirection><FeatureName>segment 6453</FeatureName></PrimaryAxis><SecondaryAxis><DefinedDirection>+Y</DefinedDirection><Source>ReferenceFrame</Source><SourceDirection>+X</SourceDirection><FeatureName></FeatureName></SecondaryAxis></Value></Frame><Frame><Id>Frame80</Id><Value><Name>L40</Name><Origin><Source>GeometricFeature</Source><FeatureName>planar surface 808</FeatureName></Origin><PrimaryAxis><DefinedDirection>+Z</DefinedDirection><Source>GeometricFeature</Source><SourceDirection>+Z</SourceDirection><FeatureName>planar surface 808</FeatureName></PrimaryAxis><SecondaryAxis><DefinedDirection>+X</DefinedDirection><Source>ReferenceFrame</Source><SourceDirection>+X</SourceDirection><FeatureName></FeatureName></SecondaryAxis></Value></Frame><Frame><Id>Frame81</Id><Value><Name>R40</Name><Origin><Source>GeometricFeature</Source><FeatureName>planar surface 80</FeatureName></Origin><PrimaryAxis><DefinedDirection>-Z</DefinedDirection><Source>GeometricFeature</Source><SourceDirection>+Z</SourceDirection><FeatureName>planar surface 80</FeatureName></PrimaryAxis><SecondaryAxis><DefinedDirection>+X</DefinedDirection><Source>ReferenceFrame</Source><SourceDirection>+X</SourceDirection><FeatureName></FeatureName></SecondaryAxis></Value></Frame><Frame><Id>Frame82</Id><Value><Name>L41</Name><Origin><Source>GeometricFeature</Source><FeatureName>planar surface 791</FeatureName></Origin><PrimaryAxis><DefinedDirection>+Z</DefinedDirection><Source>GeometricFeature</Source><SourceDirection>+Z</SourceDirection><FeatureName>planar surface 791</FeatureName></PrimaryAxis><SecondaryAxis><DefinedDirection>+X</DefinedDirection><Source>ReferenceFrame</Source><SourceDirection>+X</SourceDirection><FeatureName></FeatureName></SecondaryAxis></Value></Frame><Frame><Id>Frame83</Id><Value><Name>R41</Name><Origin><Source>GeometricFeature</Source><FeatureName>planar surface 63</FeatureName></Origin><PrimaryAxis><DefinedDirection>-Z</DefinedDirection><Source>GeometricFeature</Source><SourceDirection>+Z</SourceDirection><FeatureName>planar surface 63</FeatureName></PrimaryAxis><SecondaryAxis><DefinedDirection>+X</DefinedDirection><Source>ReferenceFrame</Source><SourceDirection>+X</SourceDirection><FeatureName></FeatureName></SecondaryAxis></Value></Frame><Frame><Id>Frame84</Id><Value><Name>L42</Name><Origin><Source>GeometricFeature</Source><FeatureName>planar surface 769</FeatureName></Origin><PrimaryAxis><DefinedDirection>+Z</DefinedDirection><Source>GeometricFeature</Source><SourceDirection>+Z</SourceDirection><FeatureName>planar surface 769</FeatureName></PrimaryAxis><SecondaryAxis><DefinedDirection>+X</DefinedDirection><Source>ReferenceFrame</Source><SourceDirection>+X</SourceDirection><FeatureName></FeatureName></SecondaryAxis></Value></Frame><Frame><Id>Frame85</Id><Value><Name>R42</Name><Origin><Source>GeometricFeature</Source><FeatureName>planar surface 41</FeatureName></Origin><PrimaryAxis><DefinedDirection>-Z</DefinedDirection><Source>GeometricFeature</Source><SourceDirection>+Z</SourceDirection><FeatureName>planar surface 41</FeatureName></PrimaryAxis><SecondaryAxis><DefinedDirection>+X</DefinedDirection><Source>ReferenceFrame</Source><SourceDirection>+X</SourceDirection><FeatureName></FeatureName></SecondaryAxis></Value></Frame><Frame><Id>Frame86</Id><Value><Name>L43</Name><Origin><Source>GeometricFeature</Source><FeatureName>segment 3140</FeatureName></Origin><PrimaryAxis><DefinedDirection>+Z</DefinedDirection><Source>GeometricFeature</Source><SourceDirection>+Z</SourceDirection><FeatureName>segment 5809</FeatureName></PrimaryAxis><SecondaryAxis><DefinedDirection>+X</DefinedDirection><Source>ReferenceFrame</Source><SourceDirection>+X</SourceDirection><FeatureName></FeatureName></SecondaryAxis></Value></Frame><Frame><Id>Frame87</Id><Value><Name>R43</Name><Origin><Source>GeometricFeature</Source><FeatureName>segment 85</FeatureName></Origin><PrimaryAxis><DefinedDirection>+Z</DefinedDirection><Source>GeometricFeature</Source><SourceDirection>+Z</SourceDirection><FeatureName>segment 2778</FeatureName></PrimaryAxis><SecondaryAxis><DefinedDirection>+X</DefinedDirection><Source>ReferenceFrame</Source><SourceDirection>+X</SourceDirection><FeatureName></FeatureName></SecondaryAxis></Value></Frame><Frame><Id>Frame88</Id><Value><Name>C1</Name><Origin><Source>GeometricFeature</Source><FeatureName>point 9476</FeatureName></Origin><PrimaryAxis><DefinedDirection>+Z</DefinedDirection><Source>GeometricFeature</Source><SourceDirection>+Z</SourceDirection><FeatureName>segment 2410</FeatureName></PrimaryAxis><SecondaryAxis><DefinedDirection>+X</DefinedDirection><Source>ReferenceFrame</Source><SourceDirection>+X</SourceDirection><FeatureName></FeatureName></SecondaryAxis></Value></Frame><Frame><Id>Frame89</Id><Value><Name>C2</Name><Origin><Source>GeometricFeature</Source><FeatureName>planar surface 1191</FeatureName></Origin><PrimaryAxis><DefinedDirection>-Z</DefinedDirection><Source>GeometricFeature</Source><SourceDirection>+Z</SourceDirection><FeatureName>planar surface 1191</FeatureName></PrimaryAxis><SecondaryAxis><DefinedDirection>+X</DefinedDirection><Source>ReferenceFrame</Source><SourceDirection>+X</SourceDirection><FeatureName></FeatureName></SecondaryAxis></Value></Frame><Frame><Id>Frame90</Id><Value><Name>Abd COM</Name><Origin><Source>CenterOfMassFrame</Source><FeatureName></FeatureName></Origin><PrimaryAxis><DefinedDirection>+Z</DefinedDirection><Source>ReferenceFrame</Source><SourceDirection>+Z</SourceDirection><FeatureName></FeatureName></PrimaryAxis><SecondaryAxis><DefinedDirection>+X</DefinedDirection><Source>ReferenceFrame</Source><SourceDirection>+X</SourceDirection><FeatureName></FeatureName></SecondaryAxis></Value></Frame></Frames>  GraphicType=FromGeometry  MarkerShape=Sphere  MarkerSize=10  GraphicVisPropType=SimpleVisualProperties  GraphicDiffuseColor=[0.5 0.5 0.5]  GraphicSpecularColor=[0.5 0.5 0.5 1.0]  GraphicAmbientColor=[0.15 0.15 0.15 1.0]  GraphicEmissiveColor=[0.0 0.0 0.0 1.0]  GraphicShininess=75  GraphicOpacity=1.0
  PS-Simulink Converter6 : nesl_utility/PS-Simulink Converter  Commented=on  PhysicalDomain=network_engine_domain  SubClassName=ps_output  LeftPortType=input  RightPortType=output  PseudoPeriodic=off  Frequencies=[]  VectorFormat=inherit  Unit=inherit  AffineConversion=off
  Rigid Transform1 : sm_lib/Frames and Transforms/Rigid Transform  Commented=on  TranslationMethod=Cartesian  TranslationStandardOffset=0  TranslationStandardOffsetUnits=m  TranslationStandardAxis=+Z  TranslationCartesianOffset=[0 116.938 1016.675]  TranslationCartesianOffsetUnits=mm  TranslationROffset=0  TranslationROffsetUnits=m  TranslationZOffset=0  TranslationZOffsetUnits=m  TranslationThetaOffset=0  TranslationThetaOffsetUnits=deg  RotationMethod=None  RotationAngleUnits=deg  RotationStandardAxis=+Z  RotationAngle=0.0  RotationArbitraryAxis=[0 0 1]  FollAlignAxisA=+X  BaseAlignAxisA=+Y  FollAlignAxisB=+Y  BaseAlignAxisB=+Z  RotationSequenceAxes=FollowerAxes  RotationSequence=XYX  RotationSequenceAngles=[0 0 0]  RotationSequenceAnglesUnits=deg  RotationMatrix=[1 0 0; 0 1 0; 0 0 1]  Quaternion=[1 0 0 0]
  Spring C1 : sm_lib/Forces and Torques/Spring and Damper Force  NaturalLength=0.1717  NaturalLengthUnits=m  SpringStiffness=K_IAP  SpringStiffnessUnits=N/m  DampingCoefficient=C_IAP  DampingCoefficientUnits=N/(m/s)  SenseForce=off
  Spring C2 : sm_lib/Forces and Torques/Spring and Damper Force  NaturalLength=0.1625  NaturalLengthUnits=m  SpringStiffness=K_IAP  SpringStiffnessUnits=N/m  DampingCoefficient=C_IAP  DampingCoefficientUnits=N/(m/s)  SenseForce=off
  Spring L1 : sm_lib/Forces and Torques/Spring and Damper Force  NaturalLength=0.04415  NaturalLengthUnits=m  SpringStiffness=K_IAP  SpringStiffnessUnits=N/m  DampingCoefficient=C_IAP  DampingCoefficientUnits=N/(m/s)  SenseForce=off
  Spring L2 : sm_lib/Forces and Torques/Spring and Damper Force  NaturalLength=0.009466  NaturalLengthUnits=m  SpringStiffness=K_IAP  SpringStiffnessUnits=N/m  DampingCoefficient=C_IAP  DampingCoefficientUnits=N/(m/s)  SenseForce=off
  Spring L3 : sm_lib/Forces and Torques/Spring and Damper Force  NaturalLength=0.02879  NaturalLengthUnits=m  SpringStiffness=K_IAP  SpringStiffnessUnits=N/m  DampingCoefficient=C_IAP  DampingCoefficientUnits=N/(m/s)  SenseForce=off
  Spring L4 : sm_lib/Forces and Torques/Spring and Damper Force  NaturalLength=0.06715  NaturalLengthUnits=m  SpringStiffness=K_IAP  SpringStiffnessUnits=N/m  DampingCoefficient=C_IAP  DampingCoefficientUnits=N/(m/s)  SenseForce=off
  Spring L5 : sm_lib/Forces and Torques/Spring and Damper Force  NaturalLength=0.09992  NaturalLengthUnits=m  SpringStiffness=K_IAP  SpringStiffnessUnits=N/m  DampingCoefficient=C_IAP  DampingCoefficientUnits=N/(m/s)  SenseForce=off
  Spring R1 : sm_lib/Forces and Torques/Spring and Damper Force  NaturalLength=0.1007  NaturalLengthUnits=m  SpringStiffness=K_IAP  SpringStiffnessUnits=N/m  DampingCoefficient=C_IAP  DampingCoefficientUnits=N/(m/s)  SenseForce=off
  Spring R10 : sm_lib/Forces and Torques/Spring and Damper Force  NaturalLength=0.1648  NaturalLengthUnits=m  SpringStiffness=K_IAP  SpringStiffnessUnits=N/m  DampingCoefficient=C_IAP  DampingCoefficientUnits=N/(m/s)  SenseForce=off
  Spring R11 : sm_lib/Forces and Torques/Spring and Damper Force  NaturalLength=0.1675  NaturalLengthUnits=m  SpringStiffness=K_IAP  SpringStiffnessUnits=N/m  DampingCoefficient=C_IAP  DampingCoefficientUnits=N/(m/s)  SenseForce=off
  Spring R12 : sm_lib/Forces and Torques/Spring and Damper Force  NaturalLength=0.1231  NaturalLengthUnits=m  SpringStiffness=K_IAP  SpringStiffnessUnits=N/m  DampingCoefficient=C_IAP  DampingCoefficientUnits=N/(m/s)  SenseForce=off
  Spring R13 : sm_lib/Forces and Torques/Spring and Damper Force  NaturalLength=0.1417  NaturalLengthUnits=m  SpringStiffness=K_IAP  SpringStiffnessUnits=N/m  DampingCoefficient=C_IAP  DampingCoefficientUnits=N/(m/s)  SenseForce=off
  Spring R14 : sm_lib/Forces and Torques/Spring and Damper Force  NaturalLength=0.1496  NaturalLengthUnits=m  SpringStiffness=K_IAP  SpringStiffnessUnits=N/m  DampingCoefficient=C_IAP  DampingCoefficientUnits=N/(m/s)  SenseForce=off
  Spring R15 : sm_lib/Forces and Torques/Spring and Damper Force  NaturalLength=0.1549  NaturalLengthUnits=m  SpringStiffness=K_IAP  SpringStiffnessUnits=N/m  DampingCoefficient=C_IAP  DampingCoefficientUnits=N/(m/s)  SenseForce=off
  Spring R16 : sm_lib/Forces and Torques/Spring and Damper Force  NaturalLength=0.1598  NaturalLengthUnits=m  SpringStiffness=K_IAP  SpringStiffnessUnits=N/m  DampingCoefficient=C_IAP  DampingCoefficientUnits=N/(m/s)  SenseForce=off
  Spring R17 : sm_lib/Forces and Torques/Spring and Damper Force  NaturalLength=0.1672  NaturalLengthUnits=m  SpringStiffness=K_IAP  SpringStiffnessUnits=N/m  DampingCoefficient=C_IAP  DampingCoefficientUnits=N/(m/s)  SenseForce=off
  Spring R18 : sm_lib/Forces and Torques/Spring and Damper Force  NaturalLength=0.1095  NaturalLengthUnits=m  SpringStiffness=K_IAP  SpringStiffnessUnits=N/m  DampingCoefficient=C_IAP  DampingCoefficientUnits=N/(m/s)  SenseForce=off
  Spring R19 : sm_lib/Forces and Torques/Spring and Damper Force  NaturalLength=0.1416  NaturalLengthUnits=m  SpringStiffness=K_IAP  SpringStiffnessUnits=N/m  DampingCoefficient=C_IAP  DampingCoefficientUnits=N/(m/s)  SenseForce=off
  Spring R2 : sm_lib/Forces and Torques/Spring and Damper Force  NaturalLength=0.137  NaturalLengthUnits=m  SpringStiffness=K_IAP  SpringStiffnessUnits=N/m  DampingCoefficient=C_IAP  DampingCoefficientUnits=N/(m/s)  SenseForce=off
  Spring R20 : sm_lib/Forces and Torques/Spring and Damper Force  NaturalLength=0.152  NaturalLengthUnits=m  SpringStiffness=K_IAP  SpringStiffnessUnits=N/m  DampingCoefficient=C_IAP  DampingCoefficientUnits=N/(m/s)  SenseForce=off
  Spring R21 : sm_lib/Forces and Torques/Spring and Damper Force  NaturalLength=0.1582  NaturalLengthUnits=m  SpringStiffness=K_IAP  SpringStiffnessUnits=N/m  DampingCoefficient=C_IAP  DampingCoefficientUnits=N/(m/s)  SenseForce=off
  Spring R22 : sm_lib/Forces and Torques/Spring and Damper Force  NaturalLength=0.1615  NaturalLengthUnits=m  SpringStiffness=K_IAP  SpringStiffnessUnits=N/m  DampingCoefficient=C_IAP  DampingCoefficientUnits=N/(m/s)  SenseForce=off
  Spring R23 : sm_lib/Forces and Torques/Spring and Damper Force  NaturalLength=0.164  NaturalLengthUnits=m  SpringStiffness=K_IAP  SpringStiffnessUnits=N/m  DampingCoefficient=C_IAP  DampingCoefficientUnits=N/(m/s)  SenseForce=off
  Spring R24 : sm_lib/Forces and Torques/Spring and Damper Force  NaturalLength=0.1273  NaturalLengthUnits=m  SpringStiffness=K_IAP  SpringStiffnessUnits=N/m  DampingCoefficient=C_IAP  DampingCoefficientUnits=N/(m/s)  SenseForce=off
  Spring R25 : sm_lib/Forces and Torques/Spring and Damper Force  NaturalLength=0.1547  NaturalLengthUnits=m  SpringStiffness=K_IAP  SpringStiffnessUnits=N/m  DampingCoefficient=C_IAP  DampingCoefficientUnits=N/(m/s)  SenseForce=off
  Spring R26 : sm_lib/Forces and Torques/Spring and Damper Force  NaturalLength=0.1602  NaturalLengthUnits=m  SpringStiffness=K_IAP  SpringStiffnessUnits=N/m  DampingCoefficient=C_IAP  DampingCoefficientUnits=N/(m/s)  SenseForce=off
  Spring R27 : sm_lib/Forces and Torques/Spring and Damper Force  NaturalLength=0.1633  NaturalLengthUnits=m  SpringStiffness=K_IAP  SpringStiffnessUnits=N/m  DampingCoefficient=C_IAP  DampingCoefficientUnits=N/(m/s)  SenseForce=off
  Spring R28 : sm_lib/Forces and Torques/Spring and Damper Force  NaturalLength=0.1629  NaturalLengthUnits=m  SpringStiffness=K_IAP  SpringStiffnessUnits=N/m  DampingCoefficient=C_IAP  DampingCoefficientUnits=N/(m/s)  SenseForce=off
  Spring R29 : sm_lib/Forces and Torques/Spring and Damper Force  NaturalLength=0.1606  NaturalLengthUnits=m  SpringStiffness=K_IAP  SpringStiffnessUnits=N/m  DampingCoefficient=C_IAP  DampingCoefficientUnits=N/(m/s)  SenseForce=off
  Spring R3 : sm_lib/Forces and Torques/Spring and Damper Force  NaturalLength=0.1116  NaturalLengthUnits=m  SpringStiffness=K_IAP  SpringStiffnessUnits=N/m  DampingCoefficient=C_IAP  DampingCoefficientUnits=N/(m/s)  SenseForce=off
  Spring R30 : sm_lib/Forces and Torques/Spring and Damper Force  NaturalLength=0.1586  NaturalLengthUnits=m  SpringStiffness=K_IAP  SpringStiffnessUnits=N/m  DampingCoefficient=C_IAP  DampingCoefficientUnits=N/(m/s)  SenseForce=off
  Spring R31 : sm_lib/Forces and Torques/Spring and Damper Force  NaturalLength=0.117  NaturalLengthUnits=m  SpringStiffness=K_IAP  SpringStiffnessUnits=N/m  DampingCoefficient=C_IAP  DampingCoefficientUnits=N/(m/s)  SenseForce=off
  Spring R32 : sm_lib/Forces and Torques/Spring and Damper Force  NaturalLength=0.1398  NaturalLengthUnits=m  SpringStiffness=K_IAP  SpringStiffnessUnits=N/m  DampingCoefficient=C_IAP  DampingCoefficientUnits=N/(m/s)  SenseForce=off
  Spring R33 : sm_lib/Forces and Torques/Spring and Damper Force  NaturalLength=0.1563  NaturalLengthUnits=m  SpringStiffness=K_IAP  SpringStiffnessUnits=N/m  DampingCoefficient=C_IAP  DampingCoefficientUnits=N/(m/s)  SenseForce=off
  Spring R34 : sm_lib/Forces and Torques/Spring and Damper Force  NaturalLength=0.1592  NaturalLengthUnits=m  SpringStiffness=K_IAP  SpringStiffnessUnits=N/m  DampingCoefficient=C_IAP  DampingCoefficientUnits=N/(m/s)  SenseForce=off
  Spring R35 : sm_lib/Forces and Torques/Spring and Damper Force  NaturalLength=0.1542  NaturalLengthUnits=m  SpringStiffness=K_IAP  SpringStiffnessUnits=N/m  DampingCoefficient=C_IAP  DampingCoefficientUnits=N/(m/s)  SenseForce=off
  Spring R36 : sm_lib/Forces and Torques/Spring and Damper Force  NaturalLength=0.1448  NaturalLengthUnits=m  SpringStiffness=K_IAP  SpringStiffnessUnits=N/m  DampingCoefficient=C_IAP  DampingCoefficientUnits=N/(m/s)  SenseForce=off
  Spring R37 : sm_lib/Forces and Torques/Spring and Damper Force  NaturalLength=0.1341  NaturalLengthUnits=m  SpringStiffness=K_IAP  SpringStiffnessUnits=N/m  DampingCoefficient=C_IAP  DampingCoefficientUnits=N/(m/s)  SenseForce=off
  Spring R38 : sm_lib/Forces and Torques/Spring and Damper Force  NaturalLength=0.1175  NaturalLengthUnits=m  SpringStiffness=K_IAP  SpringStiffnessUnits=N/m  DampingCoefficient=C_IAP  DampingCoefficientUnits=N/(m/s)  SenseForce=off
  Spring R39 : sm_lib/Forces and Torques/Spring and Damper Force  NaturalLength=0.1328  NaturalLengthUnits=m  SpringStiffness=K_IAP  SpringStiffnessUnits=N/m  DampingCoefficient=C_IAP  DampingCoefficientUnits=N/(m/s)  SenseForce=off
  Spring R4 : sm_lib/Forces and Torques/Spring and Damper Force  NaturalLength=0.1212  NaturalLengthUnits=m  SpringStiffness=K_IAP  SpringStiffnessUnits=N/m  DampingCoefficient=C_IAP  DampingCoefficientUnits=N/(m/s)  SenseForce=off
  Spring R40 : sm_lib/Forces and Torques/Spring and Damper Force  NaturalLength=0.1415  NaturalLengthUnits=m  SpringStiffness=K_IAP  SpringStiffnessUnits=N/m  DampingCoefficient=C_IAP  DampingCoefficientUnits=N/(m/s)  SenseForce=off
  Spring R41 : sm_lib/Forces and Torques/Spring and Damper Force  NaturalLength=0.1159  NaturalLengthUnits=m  SpringStiffness=K_IAP  SpringStiffnessUnits=N/m  DampingCoefficient=C_IAP  DampingCoefficientUnits=N/(m/s)  SenseForce=off
  Spring R42 : sm_lib/Forces and Torques/Spring and Damper Force  NaturalLength=0.1309  NaturalLengthUnits=m  SpringStiffness=K_IAP  SpringStiffnessUnits=N/m  DampingCoefficient=C_IAP  DampingCoefficientUnits=N/(m/s)  SenseForce=off
  Spring R43 : sm_lib/Forces and Torques/Spring and Damper Force  NaturalLength=0.1138  NaturalLengthUnits=m  SpringStiffness=K_IAP  SpringStiffnessUnits=N/m  DampingCoefficient=C_IAP  DampingCoefficientUnits=N/(m/s)  SenseForce=off
  Spring R44 : sm_lib/Forces and Torques/Spring and Damper Force  NaturalLength=0.1007  NaturalLengthUnits=m  SpringStiffness=K_IAP  SpringStiffnessUnits=N/m  DampingCoefficient=C_IAP  DampingCoefficientUnits=N/(m/s)  SenseForce=off
  Spring R45 : sm_lib/Forces and Torques/Spring and Damper Force  NaturalLength=0.1648  NaturalLengthUnits=m  SpringStiffness=K_IAP  SpringStiffnessUnits=N/m  DampingCoefficient=C_IAP  DampingCoefficientUnits=N/(m/s)  SenseForce=off
  Spring R46 : sm_lib/Forces and Torques/Spring and Damper Force  NaturalLength=0.137  NaturalLengthUnits=m  SpringStiffness=K_IAP  SpringStiffnessUnits=N/m  DampingCoefficient=C_IAP  DampingCoefficientUnits=N/(m/s)  SenseForce=off
  Spring R47 : sm_lib/Forces and Torques/Spring and Damper Force  NaturalLength=0.1116  NaturalLengthUnits=m  SpringStiffness=K_IAP  SpringStiffnessUnits=N/m  DampingCoefficient=C_IAP  DampingCoefficientUnits=N/(m/s)  SenseForce=off
  Spring R48 : sm_lib/Forces and Torques/Spring and Damper Force  NaturalLength=0.1212  NaturalLengthUnits=m  SpringStiffness=K_IAP  SpringStiffnessUnits=N/m  DampingCoefficient=C_IAP  DampingCoefficientUnits=N/(m/s)  SenseForce=off
  Spring R49 : sm_lib/Forces and Torques/Spring and Damper Force  NaturalLength=0.1124  NaturalLengthUnits=m  SpringStiffness=K_IAP  SpringStiffnessUnits=N/m  DampingCoefficient=C_IAP  DampingCoefficientUnits=N/(m/s)  SenseForce=off
  Spring R5 : sm_lib/Forces and Torques/Spring and Damper Force  NaturalLength=0.1124  NaturalLengthUnits=m  SpringStiffness=K_IAP  SpringStiffnessUnits=N/m  DampingCoefficient=C_IAP  DampingCoefficientUnits=N/(m/s)  SenseForce=off
  Spring R50 : sm_lib/Forces and Torques/Spring and Damper Force  NaturalLength=0.1308  NaturalLengthUnits=m  SpringStiffness=K_IAP  SpringStiffnessUnits=N/m  DampingCoefficient=C_IAP  DampingCoefficientUnits=N/(m/s)  SenseForce=off
  Spring R51 : sm_lib/Forces and Torques/Spring and Damper Force  NaturalLength=0.1393  NaturalLengthUnits=m  SpringStiffness=K_IAP  SpringStiffnessUnits=N/m  DampingCoefficient=C_IAP  DampingCoefficientUnits=N/(m/s)  SenseForce=off
  Spring R52 : sm_lib/Forces and Torques/Spring and Damper Force  NaturalLength=0.1486  NaturalLengthUnits=m  SpringStiffness=K_IAP  SpringStiffnessUnits=N/m  DampingCoefficient=C_IAP  DampingCoefficientUnits=N/(m/s)  SenseForce=off
  Spring R53 : sm_lib/Forces and Torques/Spring and Damper Force  NaturalLength=0.158  NaturalLengthUnits=m  SpringStiffness=K_IAP  SpringStiffnessUnits=N/m  DampingCoefficient=C_IAP  DampingCoefficientUnits=N/(m/s)  SenseForce=off
  Spring R54 : sm_lib/Forces and Torques/Spring and Damper Force  NaturalLength=0.1675  NaturalLengthUnits=m  SpringStiffness=K_IAP  SpringStiffnessUnits=N/m  DampingCoefficient=C_IAP  DampingCoefficientUnits=N/(m/s)  SenseForce=off
  Spring R55 : sm_lib/Forces and Torques/Spring and Damper Force  NaturalLength=0.1231  NaturalLengthUnits=m  SpringStiffness=K_IAP  SpringStiffnessUnits=N/m  DampingCoefficient=C_IAP  DampingCoefficientUnits=N/(m/s)  SenseForce=off
  Spring R56 : sm_lib/Forces and Torques/Spring and Damper Force  NaturalLength=0.1417  NaturalLengthUnits=m  SpringStiffness=K_IAP  SpringStiffnessUnits=N/m  DampingCoefficient=C_IAP  DampingCoefficientUnits=N/(m/s)  SenseForce=off
  Spring R57 : sm_lib/Forces and Torques/Spring and Damper Force  NaturalLength=0.1496  NaturalLengthUnits=m  SpringStiffness=K_IAP  SpringStiffnessUnits=N/m  DampingCoefficient=C_IAP  DampingCoefficientUnits=N/(m/s)  SenseForce=off
  Spring R58 : sm_lib/Forces and Torques/Spring and Damper Force  NaturalLength=0.1549  NaturalLengthUnits=m  SpringStiffness=K_IAP  SpringStiffnessUnits=N/m  DampingCoefficient=C_IAP  DampingCoefficientUnits=N/(m/s)  SenseForce=off
  Spring R59 : sm_lib/Forces and Torques/Spring and Damper Force  NaturalLength=0.1598  NaturalLengthUnits=m  SpringStiffness=K_IAP  SpringStiffnessUnits=N/m  DampingCoefficient=C_IAP  DampingCoefficientUnits=N/(m/s)  SenseForce=off
  Spring R6 : sm_lib/Forces and Torques/Spring and Damper Force  NaturalLength=0.1308  NaturalLengthUnits=m  SpringStiffness=K_IAP  SpringStiffnessUnits=N/m  DampingCoefficient=C_IAP  DampingCoefficientUnits=N/(m/s)  SenseForce=off
  Spring R60 : sm_lib/Forces and Torques/Spring and Damper Force  NaturalLength=0.1672  NaturalLengthUnits=m  SpringStiffness=K_IAP  SpringStiffnessUnits=N/m  DampingCoefficient=C_IAP  DampingCoefficientUnits=N/(m/s)  SenseForce=off
  Spring R61 : sm_lib/Forces and Torques/Spring and Damper Force  NaturalLength=0.1095  NaturalLengthUnits=m  SpringStiffness=K_IAP  SpringStiffnessUnits=N/m  DampingCoefficient=C_IAP  DampingCoefficientUnits=N/(m/s)  SenseForce=off
  Spring R62 : sm_lib/Forces and Torques/Spring and Damper Force  NaturalLength=0.1416  NaturalLengthUnits=m  SpringStiffness=K_IAP  SpringStiffnessUnits=N/m  DampingCoefficient=C_IAP  DampingCoefficientUnits=N/(m/s)  SenseForce=off
  Spring R63 : sm_lib/Forces and Torques/Spring and Damper Force  NaturalLength=0.152  NaturalLengthUnits=m  SpringStiffness=K_IAP  SpringStiffnessUnits=N/m  DampingCoefficient=C_IAP  DampingCoefficientUnits=N/(m/s)  SenseForce=off
  Spring R64 : sm_lib/Forces and Torques/Spring and Damper Force  NaturalLength=0.1582  NaturalLengthUnits=m  SpringStiffness=K_IAP  SpringStiffnessUnits=N/m  DampingCoefficient=C_IAP  DampingCoefficientUnits=N/(m/s)  SenseForce=off
  Spring R65 : sm_lib/Forces and Torques/Spring and Damper Force  NaturalLength=0.1615  NaturalLengthUnits=m  SpringStiffness=K_IAP  SpringStiffnessUnits=N/m  DampingCoefficient=C_IAP  DampingCoefficientUnits=N/(m/s)  SenseForce=off
  Spring R66 : sm_lib/Forces and Torques/Spring and Damper Force  NaturalLength=0.164  NaturalLengthUnits=m  SpringStiffness=K_IAP  SpringStiffnessUnits=N/m  DampingCoefficient=C_IAP  DampingCoefficientUnits=N/(m/s)  SenseForce=off
  Spring R67 : sm_lib/Forces and Torques/Spring and Damper Force  NaturalLength=0.1273  NaturalLengthUnits=m  SpringStiffness=K_IAP  SpringStiffnessUnits=N/m  DampingCoefficient=C_IAP  DampingCoefficientUnits=N/(m/s)  SenseForce=off
  Spring R68 : sm_lib/Forces and Torques/Spring and Damper Force  NaturalLength=0.1547  NaturalLengthUnits=m  SpringStiffness=K_IAP  SpringStiffnessUnits=N/m  DampingCoefficient=C_IAP  DampingCoefficientUnits=N/(m/s)  SenseForce=off
  Spring R69 : sm_lib/Forces and Torques/Spring and Damper Force  NaturalLength=0.1602  NaturalLengthUnits=m  SpringStiffness=K_IAP  SpringStiffnessUnits=N/m  DampingCoefficient=C_IAP  DampingCoefficientUnits=N/(m/s)  SenseForce=off
  Spring R7 : sm_lib/Forces and Torques/Spring and Damper Force  NaturalLength=0.1393  NaturalLengthUnits=m  SpringStiffness=K_IAP  SpringStiffnessUnits=N/m  DampingCoefficient=C_IAP  DampingCoefficientUnits=N/(m/s)  SenseForce=off
  Spring R70 : sm_lib/Forces and Torques/Spring and Damper Force  NaturalLength=0.1633  NaturalLengthUnits=m  SpringStiffness=K_IAP  SpringStiffnessUnits=N/m  DampingCoefficient=C_IAP  DampingCoefficientUnits=N/(m/s)  SenseForce=off
  Spring R71 : sm_lib/Forces and Torques/Spring and Damper Force  NaturalLength=0.1629  NaturalLengthUnits=m  SpringStiffness=K_IAP  SpringStiffnessUnits=N/m  DampingCoefficient=C_IAP  DampingCoefficientUnits=N/(m/s)  SenseForce=off
  Spring R72 : sm_lib/Forces and Torques/Spring and Damper Force  NaturalLength=0.1606  NaturalLengthUnits=m  SpringStiffness=K_IAP  SpringStiffnessUnits=N/m  DampingCoefficient=C_IAP  DampingCoefficientUnits=N/(m/s)  SenseForce=off
  Spring R73 : sm_lib/Forces and Torques/Spring and Damper Force  NaturalLength=0.1586  NaturalLengthUnits=m  SpringStiffness=K_IAP  SpringStiffnessUnits=N/m  DampingCoefficient=C_IAP  DampingCoefficientUnits=N/(m/s)  SenseForce=off
  Spring R74 : sm_lib/Forces and Torques/Spring and Damper Force  NaturalLength=0.117  NaturalLengthUnits=m  SpringStiffness=K_IAP  SpringStiffnessUnits=N/m  DampingCoefficient=C_IAP  DampingCoefficientUnits=N/(m/s)  SenseForce=off
  Spring R75 : sm_lib/Forces and Torques/Spring and Damper Force  NaturalLength=0.1398  NaturalLengthUnits=m  SpringStiffness=K_IAP  SpringStiffnessUnits=N/m  DampingCoefficient=C_IAP  DampingCoefficientUnits=N/(m/s)  SenseForce=off
  Spring R76 : sm_lib/Forces and Torques/Spring and Damper Force  NaturalLength=0.1563  NaturalLengthUnits=m  SpringStiffness=K_IAP  SpringStiffnessUnits=N/m  DampingCoefficient=C_IAP  DampingCoefficientUnits=N/(m/s)  SenseForce=off
  Spring R77 : sm_lib/Forces and Torques/Spring and Damper Force  NaturalLength=0.1592  NaturalLengthUnits=m  SpringStiffness=K_IAP  SpringStiffnessUnits=N/m  DampingCoefficient=C_IAP  DampingCoefficientUnits=N/(m/s)  SenseForce=off
  Spring R78 : sm_lib/Forces and Torques/Spring and Damper Force  NaturalLength=0.1542  NaturalLengthUnits=m  SpringStiffness=K_IAP  SpringStiffnessUnits=N/m  DampingCoefficient=C_IAP  DampingCoefficientUnits=N/(m/s)  SenseForce=off
  Spring R79 : sm_lib/Forces and Torques/Spring and Damper Force  NaturalLength=0.1448  NaturalLengthUnits=m  SpringStiffness=K_IAP  SpringStiffnessUnits=N/m  DampingCoefficient=C_IAP  DampingCoefficientUnits=N/(m/s)  SenseForce=off
  Spring R8 : sm_lib/Forces and Torques/Spring and Damper Force  NaturalLength=0.1486  NaturalLengthUnits=m  SpringStiffness=K_IAP  SpringStiffnessUnits=N/m  DampingCoefficient=C_IAP  DampingCoefficientUnits=N/(m/s)  SenseForce=off
  Spring R80 : sm_lib/Forces and Torques/Spring and Damper Force  NaturalLength=0.1341  NaturalLengthUnits=m  SpringStiffness=K_IAP  SpringStiffnessUnits=N/m  DampingCoefficient=C_IAP  DampingCoefficientUnits=N/(m/s)  SenseForce=off
  Spring R81 : sm_lib/Forces and Torques/Spring and Damper Force  NaturalLength=0.1175  NaturalLengthUnits=m  SpringStiffness=K_IAP  SpringStiffnessUnits=N/m  DampingCoefficient=C_IAP  DampingCoefficientUnits=N/(m/s)  SenseForce=off
  Spring R82 : sm_lib/Forces and Torques/Spring and Damper Force  NaturalLength=0.1328  NaturalLengthUnits=m  SpringStiffness=K_IAP  SpringStiffnessUnits=N/m  DampingCoefficient=C_IAP  DampingCoefficientUnits=N/(m/s)  SenseForce=off
  Spring R83 : sm_lib/Forces and Torques/Spring and Damper Force  NaturalLength=0.1415  NaturalLengthUnits=m  SpringStiffness=K_IAP  SpringStiffnessUnits=N/m  DampingCoefficient=C_IAP  DampingCoefficientUnits=N/(m/s)  SenseForce=off
  Spring R84 : sm_lib/Forces and Torques/Spring and Damper Force  NaturalLength=0.1159  NaturalLengthUnits=m  SpringStiffness=K_IAP  SpringStiffnessUnits=N/m  DampingCoefficient=C_IAP  DampingCoefficientUnits=N/(m/s)  SenseForce=off
  Spring R85 : sm_lib/Forces and Torques/Spring and Damper Force  NaturalLength=0.1309  NaturalLengthUnits=m  SpringStiffness=K_IAP  SpringStiffnessUnits=N/m  DampingCoefficient=C_IAP  DampingCoefficientUnits=N/(m/s)  SenseForce=off
  Spring R86 : sm_lib/Forces and Torques/Spring and Damper Force  NaturalLength=0.1138  NaturalLengthUnits=m  SpringStiffness=K_IAP  SpringStiffnessUnits=N/m  DampingCoefficient=C_IAP  DampingCoefficientUnits=N/(m/s)  SenseForce=off
  Spring R9 : sm_lib/Forces and Torques/Spring and Damper Force  NaturalLength=0.158  NaturalLengthUnits=m  SpringStiffness=K_IAP  SpringStiffnessUnits=N/m  DampingCoefficient=C_IAP  DampingCoefficientUnits=N/(m/s)  SenseForce=off
  Spring Sacrum1 : sm_lib/Forces and Torques/Spring and Damper Force  NaturalLength=0.2089  NaturalLengthUnits=m  SpringStiffness=11*K_IAP  SpringStiffnessUnits=N/m  DampingCoefficient=11*C_IAP  DampingCoefficientUnits=N/(m/s)  SenseForce=off
  Spring Sacrum2 : sm_lib/Forces and Torques/Spring and Damper Force  NaturalLength=0.19  NaturalLengthUnits=m  SpringStiffness=11*K_IAP  SpringStiffnessUnits=N/m  DampingCoefficient=11*C_IAP  DampingCoefficientUnits=N/(m/s)  SenseForce=off
  Spring Sacrum3 : sm_lib/Forces and Torques/Spring and Damper Force  NaturalLength=0.123  NaturalLengthUnits=m  SpringStiffness=11*K_IAP  SpringStiffnessUnits=N/m  DampingCoefficient=11*C_IAP  DampingCoefficientUnits=N/(m/s)  SenseForce=off
  Spring Sacrum4 : sm_lib/Forces and Torques/Spring and Damper Force  NaturalLength=0.123  NaturalLengthUnits=m  SpringStiffness=11*K_IAP  SpringStiffnessUnits=N/m  DampingCoefficient=11*C_IAP  DampingCoefficientUnits=N/(m/s)  SenseForce=off
  Spring Sacrum5 : sm_lib/Forces and Torques/Spring and Damper Force  NaturalLength=0.1643  NaturalLengthUnits=m  SpringStiffness=11*K_IAP  SpringStiffnessUnits=N/m  DampingCoefficient=11*C_IAP  DampingCoefficientUnits=N/(m/s)  SenseForce=off
  Spring Sacrum6 : sm_lib/Forces and Torques/Spring and Damper Force  NaturalLength=0.1643  NaturalLengthUnits=m  SpringStiffness=11*K_IAP  SpringStiffnessUnits=N/m  DampingCoefficient=11*C_IAP  DampingCoefficientUnits=N/(m/s)  SenseForce=off
  Spring Sacrum7 : sm_lib/Forces and Torques/Spring and Damper Force  NaturalLength=0.19  NaturalLengthUnits=m  SpringStiffness=11*K_IAP  SpringStiffnessUnits=N/m  DampingCoefficient=11*C_IAP  DampingCoefficientUnits=N/(m/s)  SenseForce=off
  Spring Sacrum8 : sm_lib/Forces and Torques/Spring and Damper Force  NaturalLength=0.2089  NaturalLengthUnits=m  SpringStiffness=11*K_IAP  SpringStiffnessUnits=N/m  DampingCoefficient=11*C_IAP  DampingCoefficientUnits=N/(m/s)  SenseForce=off
  Transform Sensor2 : sm_lib/Frames and Transforms/Transform Sensor  Commented=on  MeasurementFrame=World  RotationSequence=XYX  SenseAngle=off  SenseAxis=off  SenseQ=off  SenseR=off  SenseRotationSequence=off  SenseOmegaX=off  SenseOmegaY=off  SenseOmegaZ=off  SenseQDot=off  SenseRDot=off  SenseRotationSequenceDot=off  SenseAlphaX=off  SenseAlphaY=off  SenseAlphaZ=off  SenseQDDot=off  SenseRDDot=off  SenseX=off  SenseY=off  SenseZ=off  SenseRad=off  SenseAzim=off  SenseDist=on  SenseInc=off  SenseXDot=off  SenseYDot=off  SenseZDot=off  SenseRadDot=off  SenseAzimDot=off  SenseDistDot=off  SenseIncDot=off  SenseXDDot=off  SenseYDDot=off  SenseZDDot=off  SenseRadDDot=off  SenseAzimDDot=off  SenseDistDDot=off  SenseIncDDot=off
  sacrum : sm_lib/Body Elements/File Solid  ExtGeomFileName=C:\Users\siril\OneDrive\Desktop\TIM-Control\Matlab\Simscape models\CAD - with COM\SymmetricModel\sacrum.step  UnitType=FromFile  ExtGeomFileUnits=m  StepReaderType=HEX  ExportConvexHullGeometry=off  InertiaType=CalculateFromGeometry  Mass=1  MassUnits=kg  CenterOfMass=[0 0 0]  CenterOfMassUnits=m  MomentsOfInertia=[1 1 1]  MomentsOfInertiaUnits=kg*m^2  ProductsOfInertia=[0 0 0]  ProductsOfInertiaUnits=kg*m^2  BasedOnType=Density  Density=0.182  DensityUnits=g/cm^3  DoExposeReferenceFrame=on  SerializedFrames=<Frames><Frame><Id>Frame1</Id><Value><Name>To L5</Name><Origin><Source>GeometricFeature</Source><FeatureName>planar surface 14566</FeatureName></Origin><PrimaryAxis><DefinedDirection>+Z</DefinedDirection><Source>GeometricFeature</Source><SourceDirection>+Z</SourceDirection><FeatureName>planar surface 14566</FeatureName></PrimaryAxis><SecondaryAxis><DefinedDirection>+X</DefinedDirection><Source>ReferenceFrame</Source><SourceDirection>+X</SourceDirection><FeatureName></FeatureName></SecondaryAxis></Value></Frame><Frame><Id>Frame2</Id><Value><Name>To Right Abdominal Muscle</Name><Origin><Source>GeometricFeature</Source><FeatureName>planar surface 54</FeatureName></Origin><PrimaryAxis><DefinedDirection>+Z</DefinedDirection><Source>ReferenceFrame</Source><SourceDirection>+Z</SourceDirection><FeatureName></FeatureName></PrimaryAxis><SecondaryAxis><DefinedDirection>+X</DefinedDirection><Source>ReferenceFrame</Source><SourceDirection>+X</SourceDirection><FeatureName></FeatureName></SecondaryAxis></Value></Frame><Frame><Id>Frame3</Id><Value><Name>To Left Abdominal Muscle</Name><Origin><Source>GeometricFeature</Source><FeatureName>planar surface 7390</FeatureName></Origin><PrimaryAxis><DefinedDirection>+Z</DefinedDirection><Source>ReferenceFrame</Source><SourceDirection>+Z</SourceDirection><FeatureName></FeatureName></PrimaryAxis><SecondaryAxis><DefinedDirection>+X</DefinedDirection><Source>ReferenceFrame</Source><SourceDirection>+X</SourceDirection><FeatureName></FeatureName></SecondaryAxis></Value></Frame><Frame><Id>Frame4</Id><Value><Name>To Right Back Muscle</Name><Origin><Source>GeometricFeature</Source><FeatureName>planar surface 26</FeatureName></Origin><PrimaryAxis><DefinedDirection>+Z</DefinedDirection><Source>ReferenceFrame</Source><SourceDirection>+Z</SourceDirection><FeatureName></FeatureName></PrimaryAxis><SecondaryAxis><DefinedDirection>+X</DefinedDirection><Source>ReferenceFrame</Source><SourceDirection>+X</SourceDirection><FeatureName></FeatureName></SecondaryAxis></Value></Frame><Frame><Id>Frame5</Id><Value><Name>To Left Back Muscle</Name><Origin><Source>GeometricFeature</Source><FeatureName>planar surface 7362</FeatureName></Origin><PrimaryAxis><DefinedDirection>+Z</DefinedDirection><Source>ReferenceFrame</Source><SourceDirection>+Z</SourceDirection><FeatureName></FeatureName></PrimaryAxis><SecondaryAxis><DefinedDirection>+X</DefinedDirection><Source>ReferenceFrame</Source><SourceDirection>+X</SourceDirection><FeatureName></FeatureName></SecondaryAxis></Value></Frame><Frame><Id>Frame6</Id><Value><Name>To Right Transverse1 Muscle</Name><Origin><Source>GeometricFeature</Source><FeatureName>planar surface 19</FeatureName></Origin><PrimaryAxis><DefinedDirection>+Z</DefinedDirection><Source>ReferenceFrame</Source><SourceDirection>+Z</SourceDirection><FeatureName></FeatureName></PrimaryAxis><SecondaryAxis><DefinedDirection>+X</DefinedDirection><Source>ReferenceFrame</Source><SourceDirection>+X</SourceDirection><FeatureName></FeatureName></SecondaryAxis></Value></Frame><Frame><Id>Frame7</Id><Value><Name>To Right Transverse2 Muscle</Name><Origin><Source>GeometricFeature</Source><FeatureName>planar surface 5</FeatureName></Origin><PrimaryAxis><DefinedDirection>+Z</DefinedDirection><Source>ReferenceFrame</Source><SourceDirection>+Z</SourceDirection><FeatureName></FeatureName></PrimaryAxis><SecondaryAxis><DefinedDirection>+X</DefinedDirection><Source>ReferenceFrame</Source><SourceDirection>+X</SourceDirection><FeatureName></FeatureName></SecondaryAxis></Value></Frame><Frame><Id>Frame8</Id><Value><Name>To Left Transverse1 Muscle</Name><Origin><Source>GeometricFeature</Source><FeatureName>planar surface 7355</FeatureName></Origin><PrimaryAxis><DefinedDirection>+Z</DefinedDirection><Source>ReferenceFrame</Source><SourceDirection>+Z</SourceDirection><FeatureName></FeatureName></PrimaryAxis><SecondaryAxis><DefinedDirection>+X</DefinedDirection><Source>ReferenceFrame</Source><SourceDirection>+X</SourceDirection><FeatureName></FeatureName></SecondaryAxis></Value></Frame><Frame><Id>Frame9</Id><Value><Name>To Left Transverse2 Muscle</Name><Origin><Source>GeometricFeature</Source><FeatureName>planar surface 7341</FeatureName></Origin><PrimaryAxis><DefinedDirection>+Z</DefinedDirection><Source>ReferenceFrame</Source><SourceDirection>+Z</SourceDirection><FeatureName></FeatureName></PrimaryAxis><SecondaryAxis><DefinedDirection>+X</DefinedDirection><Source>ReferenceFrame</Source><SourceDirection>+X</SourceDirection><FeatureName></FeatureName></SecondaryAxis></Value></Frame><Frame><Id>Frame10</Id><Value><Name>For Plumbline Evaluation</Name><Origin><Source>GeometricFeature</Source><FeatureName>planar surface 14546</FeatureName></Origin><PrimaryAxis><DefinedDirection>+Z</DefinedDirection><Source>ReferenceFrame</Source><SourceDirection>+Z</SourceDirection><FeatureName></FeatureName></PrimaryAxis><SecondaryAxis><DefinedDirection>+X</DefinedDirection><Source>ReferenceFrame</Source><SourceDirection>+X</SourceDirection><FeatureName></FeatureName></SecondaryAxis></Value></Frame><Frame><Id>Frame11</Id><Value><Name>To Abdomen - Right</Name><Origin><Source>GeometricFeature</Source><FeatureName>planar surface 2380</FeatureName></Origin><PrimaryAxis><DefinedDirection>+Z</DefinedDirection><Source>ReferenceFrame</Source><SourceDirection>+Z</SourceDirection><FeatureName></FeatureName></PrimaryAxis><SecondaryAxis><DefinedDirection>+X</DefinedDirection><Source>ReferenceFrame</Source><SourceDirection>+X</SourceDirection><FeatureName></FeatureName></SecondaryAxis></Value></Frame><Frame><Id>Frame12</Id><Value><Name>To Abdomen - Left</Name><Origin><Source>GeometricFeature</Source><FeatureName>planar surface 9716</FeatureName></Origin><PrimaryAxis><DefinedDirection>+Z</DefinedDirection><Source>ReferenceFrame</Source><SourceDirection>+Z</SourceDirection><FeatureName></FeatureName></PrimaryAxis><SecondaryAxis><DefinedDirection>+X</DefinedDirection><Source>ReferenceFrame</Source><SourceDirection>+X</SourceDirection><FeatureName></FeatureName></SecondaryAxis></Value></Frame><Frame><Id>Frame13</Id><Value><Name>To L5 ISL</Name><Origin><Source>GeometricFeature</Source><FeatureName>point 22330</FeatureName></Origin><PrimaryAxis><DefinedDirection>+Z</DefinedDirection><Source>ReferenceFrame</Source><SourceDirection>+Z</SourceDirection><FeatureName></FeatureName></PrimaryAxis><SecondaryAxis><DefinedDirection>+X</DefinedDirection><Source>ReferenceFrame</Source><SourceDirection>+X</SourceDirection><FeatureName></FeatureName></SecondaryAxis></Value></Frame><Frame><Id>Frame14</Id><Value><Name>To L5 SSL</Name><Origin><Source>GeometricFeature</Source><FeatureName>point 44660</FeatureName></Origin><PrimaryAxis><DefinedDirection>+Z</DefinedDirection><Source>ReferenceFrame</Source><SourceDirection>+Z</SourceDirection><FeatureName></FeatureName></PrimaryAxis><SecondaryAxis><DefinedDirection>+X</DefinedDirection><Source>ReferenceFrame</Source><SourceDirection>+X</SourceDirection><FeatureName></FeatureName></SecondaryAxis></Value></Frame><Frame><Id>Frame15</Id><Value><Name>To Right L5 ITL</Name><Origin><Source>GeometricFeature</Source><FeatureName>point 13718</FeatureName></Origin><PrimaryAxis><DefinedDirection>+Z</DefinedDirection><Source>ReferenceFrame</Source><SourceDirection>+Z</SourceDirection><FeatureName></FeatureName></PrimaryAxis><SecondaryAxis><DefinedDirection>+X</DefinedDirection><Source>ReferenceFrame</Source><SourceDirection>+X</SourceDirection><FeatureName></FeatureName></SecondaryAxis></Value></Frame><Frame><Id>Frame16</Id><Value><Name>To left L5 ITL</Name><Origin><Source>GeometricFeature</Source><FeatureName>point 36305</FeatureName></Origin><PrimaryAxis><DefinedDirection>+Z</DefinedDirection><Source>ReferenceFrame</Source><SourceDirection>+Z</SourceDirection><FeatureName></FeatureName></PrimaryAxis><SecondaryAxis><DefinedDirection>+X</DefinedDirection><Source>ReferenceFrame</Source><SourceDirection>+X</SourceDirection><FeatureName></FeatureName></SecondaryAxis></Value></Frame><Frame><Id>Frame17</Id><Value><Name>Sacrum COM</Name><Origin><Source>CenterOfMassFrame</Source><FeatureName></FeatureName></Origin><PrimaryAxis><DefinedDirection>+Z</DefinedDirection><Source>ReferenceFrame</Source><SourceDirection>+Z</SourceDirection><FeatureName></FeatureName></PrimaryAxis><SecondaryAxis><DefinedDirection>+X</DefinedDirection><Source>ReferenceFrame</Source><SourceDirection>+X</SourceDirection><FeatureName></FeatureName></SecondaryAxis></Value></Frame></Frames>  GraphicType=FromGeometry  MarkerShape=Sphere  MarkerSize=10  GraphicVisPropType=SimpleVisualProperties  GraphicDiffuseColor=[0.4 1.0 0.4]  GraphicSpecularColor=[0.5 0.5 0.5 1.0]  GraphicAmbientColor=[0.15 0.15 0.15 1.0]  GraphicEmissiveColor=[0.0 0.0 0.0 1.0]  GraphicShininess=75  GraphicOpacity=1.0
  To L5 CONE : PMIOPort  Side=Right
  To L4 CONE : PMIOPort  Port=2  Side=Right
  To L2 CONE : PMIOPort  Port=3  Side=Right
  To L3 CONE : PMIOPort  Port=4  Side=Right
  To L1 CONE : PMIOPort  Port=5  Side=Right
  To L1 : PMIOPort  Port=6  Side=Left
  To Global Origin : PMIOPort  Port=7  Side=Right
  To Sacrum COM : PMIOPort  Port=8  Side=Right
  wires:
  PS-Simulink Converter6/1 -> Display/1
  connections:
  File Solid2/LConn1 -- To L1/RConn1
  Rigid Transform1/LConn1 -- To Global Origin/RConn1
  Spring R1/LConn1 -- File Solid2/RConn2
  Spring R84/RConn1 -- Spring R86/RConn1 -- Spring R85/RConn1 -- Spring R11/RConn1 -- Spring R12/RConn1 -- Spring R13/RConn1 -- Spring R14/RConn1 -- Spring R15/RConn1 -- Spring R16/RConn1 -- Spring R17/RConn1 -- Spring R18/RConn1 -- Spring R20/RConn1 -- Spring R19/RConn1 -- Spring R10/RConn1 -- Spring R31/RConn1 -- Spring R32/RConn1 -- Spring R33/RConn1 -- Spring R34/RConn1 -- Spring R35/RConn1 -- Spring R36/RConn1 -- Spring R37/RConn1 -- Spring R38/RConn1 -- Spring R39/RConn1 -- Spring R40/RConn1 -- Spring R21/RConn1 -- Spring R22/RConn1 -- Spring R23/RConn1 -- Spring R24/RConn1 -- Spring R25/RConn1 -- Spring R26/RConn1 -- Spring R27/RConn1 -- Spring R28/RConn1 -- Spring R29/RConn1 -- Spring R30/RConn1 -- Spring R43/RConn1 -- Spring R42/RConn1 -- Spring R41/RConn1 -- Spring L5/RConn1 -- Spring L4/RConn1 -- Spring L3/RConn1 -- Spring L2/RConn1 -- Spring L1/RConn1 -- Spring C2/RConn1 -- Spring C1/RConn1 -- Spring Sacrum8/LConn1 -- Spring Sacrum7/LConn1 -- Spring Sacrum6/LConn1 -- Spring Sacrum5/LConn1 -- Spring Sacrum4/RConn1 -- Spring Sacrum3/RConn1 -- Spring Sacrum2/RConn1 -- Spring Sacrum1/RConn1 -- Rigid Transform1/RConn1 -- File Solid/LConn1 -- Transform Sensor2/RConn1 -- Spring R9/RConn1 -- Spring R8/RConn1 -- Spring R7/RConn1 -- Spring R6/RConn1 -- Spring R1/RConn1 -- Spring R2/RConn1 -- Spring R3/RConn1 -- Spring R4/RConn1 -- Spring R5/RConn1 -- Spring R45/RConn1 -- Spring R53/RConn1 -- Spring R52/RConn1 -- Spring R51/RConn1 -- Spring R50/RConn1 -- Spring R49/RConn1 -- Spring R48/RConn1 -- Spring R47/RConn1 -- Spring R46/RConn1 -- Spring R44/RConn1 -- Spring R54/RConn1 -- Spring R55/RConn1 -- Spring R56/RConn1 -- Spring R57/RConn1 -- Spring R58/RConn1 -- Spring R59/RConn1 -- Spring R60/RConn1 -- Spring R61/RConn1 -- Spring R63/RConn1 -- Spring R62/RConn1 -- Spring R83/RConn1 -- Spring R82/RConn1 -- Spring R81/RConn1 -- Spring R80/RConn1 -- Spring R79/RConn1 -- Spring R78/RConn1 -- Spring R77/RConn1 -- Spring R76/RConn1 -- Spring R75/RConn1 -- Spring R74/RConn1 -- Spring R73/RConn1 -- Spring R72/RConn1 -- Spring R71/RConn1 -- Spring R70/RConn1 -- Spring R69/RConn1 -- Spring R68/RConn1 -- Spring R67/RConn1 -- Spring R66/RConn1 -- Spring R65/RConn1 -- Spring R64/RConn1
  Spring R2/LConn1 -- File Solid2/RConn3
  Spring R3/LConn1 -- File Solid2/RConn4
  Spring R4/LConn1 -- File Solid2/RConn5
  PS-Simulink Converter6/LConn1 -- Transform Sensor2/RConn2
  Spring R5/LConn1 -- File Solid2/RConn6
  Spring R6/LConn1 -- File Solid2/RConn7
  Spring R7/LConn1 -- File Solid2/RConn8
  Spring R8/LConn1 -- File Solid2/RConn9
  Spring R9/LConn1 -- File Solid2/RConn10
  Spring R10/LConn1 -- File Solid2/RConn11
  Spring R11/LConn1 -- File Solid2/RConn12
  Spring R12/LConn1 -- File Solid2/RConn13
  Spring R13/LConn1 -- File Solid2/RConn14
  Spring R14/LConn1 -- File Solid2/RConn15
  Spring R15/LConn1 -- File Solid2/RConn16
  Spring R16/LConn1 -- File Solid2/RConn17
  Spring R17/LConn1 -- File Solid2/RConn18
  Spring R18/LConn1 -- File Solid2/RConn19
  Spring R19/LConn1 -- File Solid2/RConn20
  Spring R20/LConn1 -- File Solid2/RConn21
  Spring R21/LConn1 -- File Solid2/RConn22
  Spring R22/LConn1 -- File Solid2/RConn23
  Spring R23/LConn1 -- File Solid2/RConn24
  Spring R24/LConn1 -- File Solid2/RConn25
  Spring R25/LConn1 -- File Solid2/RConn26
  Spring R26/LConn1 -- File Solid2/RConn27
  Spring R27/LConn1 -- File Solid2/RConn28
  Spring R28/LConn1 -- File Solid2/RConn29
  Spring R29/LConn1 -- File Solid2/RConn30
  Spring R30/LConn1 -- File Solid2/RConn31
  Spring R31/LConn1 -- File Solid2/RConn32
  Spring R32/LConn1 -- File Solid2/RConn33
  Spring R33/LConn1 -- File Solid2/RConn34
  Spring R34/LConn1 -- File Solid2/RConn35
  Spring R35/LConn1 -- File Solid2/RConn36
  Spring R36/LConn1 -- File Solid2/RConn37
  Spring R37/LConn1 -- File Solid2/RConn38
  Spring R38/LConn1 -- File Solid2/RConn39
  Spring R39/LConn1 -- File Solid2/RConn40
  Spring R40/LConn1 -- File Solid2/RConn41
  Spring R41/LConn1 -- File Solid2/RConn42
  Spring R42/LConn1 -- File Solid2/RConn43
  Spring R43/LConn1 -- File Solid2/RConn44
  Spring C1/LConn1 -- File Solid2/LConn45
  Spring C2/LConn1 -- File Solid2/RConn45
  Spring R48/LConn1 -- File Solid2/LConn5
  Spring R44/LConn1 -- File Solid2/LConn2
  Spring R50/LConn1 -- File Solid2/LConn7
  Spring R45/LConn1 -- File Solid2/LConn11
  Spring R49/LConn1 -- File Solid2/LConn6
  Spring R47/LConn1 -- File Solid2/LConn4
  Spring R53/LConn1 -- File Solid2/LConn10
  Spring R52/LConn1 -- File Solid2/LConn9
  Spring R51/LConn1 -- File Solid2/LConn8
  Spring R46/LConn1 -- File Solid2/LConn3
  Spring R59/LConn1 -- File Solid2/LConn17
  Spring R63/LConn1 -- File Solid2/LConn21
  Spring R61/LConn1 -- File Solid2/LConn19
  Spring R60/LConn1 -- File Solid2/LConn18
  Spring R55/LConn1 -- File Solid2/LConn13
  Spring R58/LConn1 -- File Solid2/LConn16
  Spring R62/LConn1 -- File Solid2/LConn20
  Spring R54/LConn1 -- File Solid2/LConn12
  Spring R56/LConn1 -- File Solid2/LConn14
  Spring R57/LConn1 -- File Solid2/LConn15
  Spring R64/LConn1 -- File Solid2/LConn22
  Spring R65/LConn1 -- File Solid2/LConn23
  Spring R66/LConn1 -- File Solid2/LConn24
  Spring R67/LConn1 -- File Solid2/LConn25
  Spring R68/LConn1 -- File Solid2/LConn26
  Spring R69/LConn1 -- File Solid2/LConn27
  Spring R70/LConn1 -- File Solid2/LConn28
  Spring R71/LConn1 -- File Solid2/LConn29
  Spring R72/LConn1 -- File Solid2/LConn30
  Spring R73/LConn1 -- File Solid2/LConn31
  Spring R74/LConn1 -- File Solid2/LConn32
  Spring R75/LConn1 -- File Solid2/LConn33
  Spring R76/LConn1 -- File Solid2/LConn34
  Spring R77/LConn1 -- File Solid2/LConn35
  Spring R78/LConn1 -- File Solid2/LConn36
  Spring R79/LConn1 -- File Solid2/LConn37
  Spring R80/LConn1 -- File Solid2/LConn38
  Spring R81/LConn1 -- File Solid2/LConn39
  Spring R82/LConn1 -- File Solid2/LConn40
  Spring R83/LConn1 -- File Solid2/LConn41
  Spring R84/LConn1 -- File Solid2/LConn42
  Spring R85/LConn1 -- File Solid2/LConn43
  Spring R86/LConn1 -- File Solid2/LConn44
  Spring L1/LConn1 -- To L1 CONE/RConn1
  Spring L2/LConn1 -- To L2 CONE/RConn1
  Spring L3/LConn1 -- To L3 CONE/RConn1
  Spring L4/LConn1 -- To L4 CONE/RConn1
  Spring L5/LConn1 -- To L5 CONE/RConn1
  To Sacrum COM/RConn1 -- sacrum/RConn9
  Spring Sacrum1/LConn1 -- sacrum/LConn2
  Spring Sacrum2/LConn1 -- sacrum/LConn3
  Spring Sacrum3/LConn1 -- sacrum/LConn4
  Spring Sacrum4/LConn1 -- sacrum/LConn5
  Spring Sacrum5/RConn1 -- sacrum/RConn5
  Spring Sacrum6/RConn1 -- sacrum/RConn4
  Spring Sacrum7/RConn1 -- sacrum/RConn3
  Spring Sacrum8/RConn1 -- sacrum/RConn2
